simulink model "model"  (R2014a)
(part 3 of 4)

  bus249 : powerlib/Measurements/Load Flow Bus  LConnTagsString=a  ID=bus249  Vbase=150000  Vref=1  Vangle=0  VLF=1  angleLF=0
      settings: AttributesFormatString=|
      | %<ID>
      | %<Vbase>V
      | %<VLF>pu
      | %<angleLF>deg.
      | %<Name>
  bus25 : powerlib/Measurements/Load Flow Bus  LConnTagsString=a  ID=bus25  Vbase=150000  Vref=1  Vangle=0  VLF=1  angleLF=0
      settings: AttributesFormatString=|
      | %<ID>
      | %<Vbase>V
      | %<VLF>pu
      | %<angleLF>deg.
      | %<Name>
  bus250 : powerlib/Measurements/Load Flow Bus  LConnTagsString=a  ID=bus250  Vbase=150000  Vref=1  Vangle=0  VLF=1  angleLF=0
      settings: AttributesFormatString=|
      | %<ID>
      | %<Vbase>V
      | %<VLF>pu
      | %<angleLF>deg.
      | %<Name>
  bus251 : powerlib/Measurements/Load Flow Bus  LConnTagsString=a  ID=bus251  Vbase=150000  Vref=1  Vangle=0  VLF=1  angleLF=0
      settings: AttributesFormatString=|
      | %<ID>
      | %<Vbase>V
      | %<VLF>pu
      | %<angleLF>deg.
      | %<Name>
  bus252 : powerlib/Measurements/Load Flow Bus  LConnTagsString=a  ID=bus252  Vbase=150000  Vref=1  Vangle=0  VLF=1  angleLF=0
      settings: AttributesFormatString=|
      | %<ID>
      | %<Vbase>V
      | %<VLF>pu
      | %<angleLF>deg.
      | %<Name>
  bus253 : powerlib/Measurements/Load Flow Bus  LConnTagsString=a  ID=bus253  Vbase=150000  Vref=1  Vangle=0  VLF=1  angleLF=0
      settings: AttributesFormatString=|
      | %<ID>
      | %<Vbase>V
      | %<VLF>pu
      | %<angleLF>deg.
      | %<Name>
  bus254 : powerlib/Measurements/Load Flow Bus  LConnTagsString=a  ID=bus254  Vbase=150000  Vref=1  Vangle=0  VLF=1  angleLF=0
      settings: AttributesFormatString=|
      | %<ID>
      | %<Vbase>V
      | %<VLF>pu
      | %<angleLF>deg.
      | %<Name>
  bus255 : powerlib/Measurements/Load Flow Bus  LConnTagsString=a  ID=bus255  Vbase=150000  Vref=1  Vangle=0  VLF=1  angleLF=0
      settings: AttributesFormatString=|
      | %<ID>
      | %<Vbase>V
      | %<VLF>pu
      | %<angleLF>deg.
      | %<Name>
  bus256 : powerlib/Measurements/Load Flow Bus  LConnTagsString=a  ID=bus256  Vbase=150000  Vref=1  Vangle=0  VLF=1  angleLF=0
      settings: AttributesFormatString=|
      | %<ID>
      | %<Vbase>V
      | %<VLF>pu
      | %<angleLF>deg.
      | %<Name>
  bus257 : powerlib/Measurements/Load Flow Bus  LConnTagsString=a  ID=bus257  Vbase=150000  Vref=1  Vangle=0  VLF=1  angleLF=0
      settings: AttributesFormatString=|
      | %<ID>
      | %<Vbase>V
      | %<VLF>pu
      | %<angleLF>deg.
      | %<Name>
  bus258 : powerlib/Measurements/Load Flow Bus  LConnTagsString=a  ID=bus258  Vbase=150000  Vref=1  Vangle=0  VLF=1  angleLF=0
      settings: AttributesFormatString=|
      | %<ID>
      | %<Vbase>V
      | %<VLF>pu
      | %<angleLF>deg.
      | %<Name>
  bus259 : powerlib/Measurements/Load Flow Bus  LConnTagsString=a  ID=bus259  Vbase=150000  Vref=1  Vangle=0  VLF=1  angleLF=0
      settings: AttributesFormatString=|
      | %<ID>
      | %<Vbase>V
      | %<VLF>pu
      | %<angleLF>deg.
      | %<Name>
  bus26 : powerlib/Measurements/Load Flow Bus  LConnTagsString=a  ID=bus26  Vbase=150000  Vref=1  Vangle=0  VLF=1  angleLF=0
      settings: AttributesFormatString=|
      | %<ID>
      | %<Vbase>V
      | %<VLF>pu
      | %<angleLF>deg.
      | %<Name>
  bus260 : powerlib/Measurements/Load Flow Bus  LConnTagsString=a  ID=bus260  Vbase=150000  Vref=1  Vangle=0  VLF=1  angleLF=0
      settings: AttributesFormatString=|
      | %<ID>
      | %<Vbase>V
      | %<VLF>pu
      | %<angleLF>deg.
      | %<Name>
  bus261 : powerlib/Measurements/Load Flow Bus  LConnTagsString=a  ID=bus261  Vbase=150000  Vref=1  Vangle=0  VLF=1  angleLF=0
      settings: AttributesFormatString=|
      | %<ID>
      | %<Vbase>V
      | %<VLF>pu
      | %<angleLF>deg.
      | %<Name>
  bus262 : powerlib/Measurements/Load Flow Bus  LConnTagsString=a  ID=bus262  Vbase=150000  Vref=1  Vangle=0  VLF=1  angleLF=0
      settings: AttributesFormatString=|
      | %<ID>
      | %<Vbase>V
      | %<VLF>pu
      | %<angleLF>deg.
      | %<Name>
  bus263 : powerlib/Measurements/Load Flow Bus  LConnTagsString=a  ID=bus263  Vbase=150000  Vref=1  Vangle=0  VLF=1  angleLF=0
      settings: AttributesFormatString=|
      | %<ID>
      | %<Vbase>V
      | %<VLF>pu
      | %<angleLF>deg.
      | %<Name>
  bus264 : powerlib/Measurements/Load Flow Bus  LConnTagsString=a  ID=bus264  Vbase=150000  Vref=1  Vangle=0  VLF=1  angleLF=0
      settings: AttributesFormatString=|
      | %<ID>
      | %<Vbase>V
      | %<VLF>pu
      | %<angleLF>deg.
      | %<Name>
  bus265 : powerlib/Measurements/Load Flow Bus  LConnTagsString=a  ID=bus265  Vbase=150000  Vref=1  Vangle=0  VLF=1  angleLF=0
      settings: AttributesFormatString=|
      | %<ID>
      | %<Vbase>V
      | %<VLF>pu
      | %<angleLF>deg.
      | %<Name>
  bus266 : powerlib/Measurements/Load Flow Bus  LConnTagsString=a  ID=bus266  Vbase=150000  Vref=1  Vangle=0  VLF=1  angleLF=0
      settings: AttributesFormatString=|
      | %<ID>
      | %<Vbase>V
      | %<VLF>pu
      | %<angleLF>deg.
      | %<Name>
  bus267 : powerlib/Measurements/Load Flow Bus  LConnTagsString=a  ID=bus267  Vbase=150000  Vref=1  Vangle=0  VLF=1  angleLF=0
      settings: AttributesFormatString=|
      | %<ID>
      | %<Vbase>V
      | %<VLF>pu
      | %<angleLF>deg.
      | %<Name>
  bus268 : powerlib/Measurements/Load Flow Bus  LConnTagsString=a  ID=bus268  Vbase=150000  Vref=1  Vangle=0  VLF=1  angleLF=0
      settings: AttributesFormatString=|
      | %<ID>
      | %<Vbase>V
      | %<VLF>pu
      | %<angleLF>deg.
      | %<Name>
  bus269 : powerlib/Measurements/Load Flow Bus  LConnTagsString=a  ID=bus269  Vbase=150000  Vref=1  Vangle=0  VLF=1  angleLF=0
      settings: AttributesFormatString=|
      | %<ID>
      | %<Vbase>V
      | %<VLF>pu
      | %<angleLF>deg.
      | %<Name>
  bus27 : powerlib/Measurements/Load Flow Bus  LConnTagsString=a  ID=bus27  Vbase=150000  Vref=1  Vangle=0  VLF=1  angleLF=0
      settings: AttributesFormatString=|
      | %<ID>
      | %<Vbase>V
      | %<VLF>pu
      | %<angleLF>deg.
      | %<Name>
  bus270 : powerlib/Measurements/Load Flow Bus  LConnTagsString=a  ID=bus270  Vbase=150000  Vref=1  Vangle=0  VLF=1  angleLF=0
      settings: AttributesFormatString=|
      | %<ID>
      | %<Vbase>V
      | %<VLF>pu
      | %<angleLF>deg.
      | %<Name>
  bus271 : powerlib/Measurements/Load Flow Bus  LConnTagsString=a  ID=bus271  Vbase=150000  Vref=1  Vangle=0  VLF=1  angleLF=0
      settings: AttributesFormatString=|
      | %<ID>
      | %<Vbase>V
      | %<VLF>pu
      | %<angleLF>deg.
      | %<Name>
  bus272 : powerlib/Measurements/Load Flow Bus  LConnTagsString=a  ID=bus272  Vbase=150000  Vref=1  Vangle=0  VLF=1  angleLF=0
      settings: AttributesFormatString=|
      | %<ID>
      | %<Vbase>V
      | %<VLF>pu
      | %<angleLF>deg.
      | %<Name>
  bus273 : powerlib/Measurements/Load Flow Bus  LConnTagsString=a  ID=bus273  Vbase=150000  Vref=1  Vangle=0  VLF=1  angleLF=0
      settings: AttributesFormatString=|
      | %<ID>
      | %<Vbase>V
      | %<VLF>pu
      | %<angleLF>deg.
      | %<Name>
  bus274 : powerlib/Measurements/Load Flow Bus  LConnTagsString=a  ID=bus274  Vbase=150000  Vref=1  Vangle=0  VLF=1  angleLF=0
      settings: AttributesFormatString=|
      | %<ID>
      | %<Vbase>V
      | %<VLF>pu
      | %<angleLF>deg.
      | %<Name>
  bus275 : powerlib/Measurements/Load Flow Bus  LConnTagsString=a  ID=bus275  Vbase=150000  Vref=1  Vangle=0  VLF=1  angleLF=0
      settings: AttributesFormatString=|
      | %<ID>
      | %<Vbase>V
      | %<VLF>pu
      | %<angleLF>deg.
      | %<Name>
  bus276 : powerlib/Measurements/Load Flow Bus  LConnTagsString=a  ID=bus276  Vbase=150000  Vref=1  Vangle=0  VLF=1  angleLF=0
      settings: AttributesFormatString=|
      | %<ID>
      | %<Vbase>V
      | %<VLF>pu
      | %<angleLF>deg.
      | %<Name>
  bus277 : powerlib/Measurements/Load Flow Bus  LConnTagsString=a  ID=bus277  Vbase=150000  Vref=1  Vangle=0  VLF=1  angleLF=0
      settings: AttributesFormatString=|
      | %<ID>
      | %<Vbase>V
      | %<VLF>pu
      | %<angleLF>deg.
      | %<Name>
  bus278 : powerlib/Measurements/Load Flow Bus  LConnTagsString=a  ID=bus278  Vbase=150000  Vref=1  Vangle=0  VLF=1  angleLF=0
      settings: AttributesFormatString=|
      | %<ID>
      | %<Vbase>V
      | %<VLF>pu
      | %<angleLF>deg.
      | %<Name>
  bus279 : powerlib/Measurements/Load Flow Bus  LConnTagsString=a  ID=bus279  Vbase=150000  Vref=1  Vangle=0  VLF=1  angleLF=0
      settings: AttributesFormatString=|
      | %<ID>
      | %<Vbase>V
      | %<VLF>pu
      | %<angleLF>deg.
      | %<Name>
  bus28 : powerlib/Measurements/Load Flow Bus  LConnTagsString=a  ID=bus28  Vbase=150000  Vref=1  Vangle=0  VLF=1  angleLF=0
      settings: AttributesFormatString=|
      | %<ID>
      | %<Vbase>V
      | %<VLF>pu
      | %<angleLF>deg.
      | %<Name>
  bus280 : powerlib/Measurements/Load Flow Bus  LConnTagsString=a  ID=bus280  Vbase=150000  Vref=1  Vangle=0  VLF=1  angleLF=0
      settings: AttributesFormatString=|
      | %<ID>
      | %<Vbase>V
      | %<VLF>pu
      | %<angleLF>deg.
      | %<Name>
  bus281 : powerlib/Measurements/Load Flow Bus  LConnTagsString=a  ID=bus281  Vbase=150000  Vref=1  Vangle=0  VLF=1  angleLF=0
      settings: AttributesFormatString=|
      | %<ID>
      | %<Vbase>V
      | %<VLF>pu
      | %<angleLF>deg.
      | %<Name>
  bus282 : powerlib/Measurements/Load Flow Bus  LConnTagsString=a  ID=bus282  Vbase=150000  Vref=1  Vangle=0  VLF=1  angleLF=0
      settings: AttributesFormatString=|
      | %<ID>
      | %<Vbase>V
      | %<VLF>pu
      | %<angleLF>deg.
      | %<Name>
  bus283 : powerlib/Measurements/Load Flow Bus  LConnTagsString=a  ID=bus283  Vbase=150000  Vref=1  Vangle=0  VLF=1  angleLF=0
      settings: AttributesFormatString=|
      | %<ID>
      | %<Vbase>V
      | %<VLF>pu
      | %<angleLF>deg.
      | %<Name>
  bus284 : powerlib/Measurements/Load Flow Bus  LConnTagsString=a  ID=bus284  Vbase=150000  Vref=1  Vangle=0  VLF=1  angleLF=0
      settings: AttributesFormatString=|
      | %<ID>
      | %<Vbase>V
      | %<VLF>pu
      | %<angleLF>deg.
      | %<Name>
  bus285 : powerlib/Measurements/Load Flow Bus  LConnTagsString=a  ID=bus285  Vbase=150000  Vref=1  Vangle=0  VLF=1  angleLF=0
      settings: AttributesFormatString=|
      | %<ID>
      | %<Vbase>V
      | %<VLF>pu
      | %<angleLF>deg.
      | %<Name>
  bus286 : powerlib/Measurements/Load Flow Bus  LConnTagsString=a  ID=bus286  Vbase=150000  Vref=1  Vangle=0  VLF=1  angleLF=0
      settings: AttributesFormatString=|
      | %<ID>
      | %<Vbase>V
      | %<VLF>pu
      | %<angleLF>deg.
      | %<Name>
  bus287 : powerlib/Measurements/Load Flow Bus  LConnTagsString=a  ID=bus287  Vbase=150000  Vref=1  Vangle=0  VLF=1  angleLF=0
      settings: AttributesFormatString=|
      | %<ID>
      | %<Vbase>V
      | %<VLF>pu
      | %<angleLF>deg.
      | %<Name>
  bus288 : powerlib/Measurements/Load Flow Bus  LConnTagsString=a  ID=bus288  Vbase=150000  Vref=1  Vangle=0  VLF=1  angleLF=0
      settings: AttributesFormatString=|
      | %<ID>
      | %<Vbase>V
      | %<VLF>pu
      | %<angleLF>deg.
      | %<Name>
  bus289 : powerlib/Measurements/Load Flow Bus  LConnTagsString=a  ID=bus289  Vbase=150000  Vref=1  Vangle=0  VLF=1  angleLF=0
      settings: AttributesFormatString=|
      | %<ID>
      | %<Vbase>V
      | %<VLF>pu
      | %<angleLF>deg.
      | %<Name>
  bus29 : powerlib/Measurements/Load Flow Bus  LConnTagsString=a  ID=bus29  Vbase=150000  Vref=1  Vangle=0  VLF=1  angleLF=0
      settings: AttributesFormatString=|
      | %<ID>
      | %<Vbase>V
      | %<VLF>pu
      | %<angleLF>deg.
      | %<Name>
  bus290 : powerlib/Measurements/Load Flow Bus  LConnTagsString=a  ID=bus290  Vbase=150000  Vref=1  Vangle=0  VLF=1  angleLF=0
      settings: AttributesFormatString=|
      | %<ID>
      | %<Vbase>V
      | %<VLF>pu
      | %<angleLF>deg.
      | %<Name>
  bus291 : powerlib/Measurements/Load Flow Bus  LConnTagsString=a  ID=bus291  Vbase=150000  Vref=1  Vangle=0  VLF=1  angleLF=0
      settings: AttributesFormatString=|
      | %<ID>
      | %<Vbase>V
      | %<VLF>pu
      | %<angleLF>deg.
      | %<Name>
  bus292 : powerlib/Measurements/Load Flow Bus  LConnTagsString=a  ID=bus292  Vbase=150000  Vref=1  Vangle=0  VLF=1  angleLF=0
      settings: AttributesFormatString=|
      | %<ID>
      | %<Vbase>V
      | %<VLF>pu
      | %<angleLF>deg.
      | %<Name>
  bus293 : powerlib/Measurements/Load Flow Bus  LConnTagsString=a  ID=bus293  Vbase=150000  Vref=1  Vangle=0  VLF=1  angleLF=0
      settings: AttributesFormatString=|
      | %<ID>
      | %<Vbase>V
      | %<VLF>pu
      | %<angleLF>deg.
      | %<Name>
  bus294 : powerlib/Measurements/Load Flow Bus  LConnTagsString=a  ID=bus294  Vbase=150000  Vref=1  Vangle=0  VLF=1  angleLF=0
      settings: AttributesFormatString=|
      | %<ID>
      | %<Vbase>V
      | %<VLF>pu
      | %<angleLF>deg.
      | %<Name>
  bus295 : powerlib/Measurements/Load Flow Bus  LConnTagsString=a  ID=bus295  Vbase=150000  Vref=1  Vangle=0  VLF=1  angleLF=0
      settings: AttributesFormatString=|
      | %<ID>
      | %<Vbase>V
      | %<VLF>pu
      | %<angleLF>deg.
      | %<Name>
  bus296 : powerlib/Measurements/Load Flow Bus  LConnTagsString=a  ID=bus296  Vbase=150000  Vref=1  Vangle=0  VLF=1  angleLF=0
      settings: AttributesFormatString=|
      | %<ID>
      | %<Vbase>V
      | %<VLF>pu
      | %<angleLF>deg.
      | %<Name>
  bus297 : powerlib/Measurements/Load Flow Bus  LConnTagsString=a  ID=bus297  Vbase=150000  Vref=1  Vangle=0  VLF=1  angleLF=0
      settings: AttributesFormatString=|
      | %<ID>
      | %<Vbase>V
      | %<VLF>pu
      | %<angleLF>deg.
      | %<Name>
  bus298 : powerlib/Measurements/Load Flow Bus  LConnTagsString=a  ID=bus298  Vbase=150000  Vref=1  Vangle=0  VLF=1  angleLF=0
      settings: AttributesFormatString=|
      | %<ID>
      | %<Vbase>V
      | %<VLF>pu
      | %<angleLF>deg.
      | %<Name>
  bus299 : powerlib/Measurements/Load Flow Bus  LConnTagsString=a  ID=bus299  Vbase=150000  Vref=1  Vangle=0  VLF=1  angleLF=0
      settings: AttributesFormatString=|
      | %<ID>
      | %<Vbase>V
      | %<VLF>pu
      | %<angleLF>deg.
      | %<Name>
  bus3 : powerlib/Measurements/Load Flow Bus  LConnTagsString=a  ID=bus3  Vbase=150000  Vref=1  Vangle=0  VLF=1  angleLF=0
      settings: AttributesFormatString=|
      | %<ID>
      | %<Vbase>V
      | %<VLF>pu
      | %<angleLF>deg.
      | %<Name>
  bus30 : powerlib/Measurements/Load Flow Bus  LConnTagsString=a  ID=bus30  Vbase=150000  Vref=1  Vangle=0  VLF=1  angleLF=0
      settings: AttributesFormatString=|
      | %<ID>
      | %<Vbase>V
      | %<VLF>pu
      | %<angleLF>deg.
      | %<Name>
  bus300 : powerlib/Measurements/Load Flow Bus  LConnTagsString=a  ID=bus300  Vbase=150000  Vref=1  Vangle=0  VLF=1  angleLF=0
      settings: AttributesFormatString=|
      | %<ID>
      | %<Vbase>V
      | %<VLF>pu
      | %<angleLF>deg.
      | %<Name>
  bus301 : powerlib/Measurements/Load Flow Bus  LConnTagsString=a  ID=bus301  Vbase=150000  Vref=1  Vangle=0  VLF=1  angleLF=0
      settings: AttributesFormatString=|
      | %<ID>
      | %<Vbase>V
      | %<VLF>pu
      | %<angleLF>deg.
      | %<Name>
  bus302 : powerlib/Measurements/Load Flow Bus  LConnTagsString=a  ID=bus302  Vbase=150000  Vref=1  Vangle=0  VLF=1  angleLF=0
      settings: AttributesFormatString=|
      | %<ID>
      | %<Vbase>V
      | %<VLF>pu
      | %<angleLF>deg.
      | %<Name>
  bus303 : powerlib/Measurements/Load Flow Bus  LConnTagsString=a  ID=bus303  Vbase=150000  Vref=1  Vangle=0  VLF=1  angleLF=0
      settings: AttributesFormatString=|
      | %<ID>
      | %<Vbase>V
      | %<VLF>pu
      | %<angleLF>deg.
      | %<Name>
  bus304 : powerlib/Measurements/Load Flow Bus  LConnTagsString=a  ID=bus304  Vbase=150000  Vref=1  Vangle=0  VLF=1  angleLF=0
      settings: AttributesFormatString=|
      | %<ID>
      | %<Vbase>V
      | %<VLF>pu
      | %<angleLF>deg.
      | %<Name>
  bus305 : powerlib/Measurements/Load Flow Bus  LConnTagsString=a  ID=bus305  Vbase=150000  Vref=1  Vangle=0  VLF=1  angleLF=0
      settings: AttributesFormatString=|
      | %<ID>
      | %<Vbase>V
      | %<VLF>pu
      | %<angleLF>deg.
      | %<Name>
  bus306 : powerlib/Measurements/Load Flow Bus  LConnTagsString=a  ID=bus306  Vbase=150000  Vref=1  Vangle=0  VLF=1  angleLF=0
      settings: AttributesFormatString=|
      | %<ID>
      | %<Vbase>V
      | %<VLF>pu
      | %<angleLF>deg.
      | %<Name>
  bus307 : powerlib/Measurements/Load Flow Bus  LConnTagsString=a  ID=bus307  Vbase=150000  Vref=1  Vangle=0  VLF=1  angleLF=0
      settings: AttributesFormatString=|
      | %<ID>
      | %<Vbase>V
      | %<VLF>pu
      | %<angleLF>deg.
      | %<Name>
  bus308 : powerlib/Measurements/Load Flow Bus  LConnTagsString=a  ID=bus308  Vbase=150000  Vref=1  Vangle=0  VLF=1  angleLF=0
      settings: AttributesFormatString=|
      | %<ID>
      | %<Vbase>V
      | %<VLF>pu
      | %<angleLF>deg.
      | %<Name>
  bus309 : powerlib/Measurements/Load Flow Bus  LConnTagsString=a  ID=bus309  Vbase=150000  Vref=1  Vangle=0  VLF=1  angleLF=0
      settings: AttributesFormatString=|
      | %<ID>
      | %<Vbase>V
      | %<VLF>pu
      | %<angleLF>deg.
      | %<Name>
  bus31 : powerlib/Measurements/Load Flow Bus  LConnTagsString=a  ID=bus31  Vbase=150000  Vref=1  Vangle=0  VLF=1  angleLF=0
      settings: AttributesFormatString=|
      | %<ID>
      | %<Vbase>V
      | %<VLF>pu
      | %<angleLF>deg.
      | %<Name>
  bus310 : powerlib/Measurements/Load Flow Bus  LConnTagsString=a  ID=bus310  Vbase=150000  Vref=1  Vangle=0  VLF=1  angleLF=0
      settings: AttributesFormatString=|
      | %<ID>
      | %<Vbase>V
      | %<VLF>pu
      | %<angleLF>deg.
      | %<Name>
  bus311 : powerlib/Measurements/Load Flow Bus  LConnTagsString=a  ID=bus311  Vbase=150000  Vref=1  Vangle=0  VLF=1  angleLF=0
      settings: AttributesFormatString=|
      | %<ID>
      | %<Vbase>V
      | %<VLF>pu
      | %<angleLF>deg.
      | %<Name>
  bus312 : powerlib/Measurements/Load Flow Bus  LConnTagsString=a  ID=bus312  Vbase=150000  Vref=1  Vangle=0  VLF=1  angleLF=0
      settings: AttributesFormatString=|
      | %<ID>
      | %<Vbase>V
      | %<VLF>pu
      | %<angleLF>deg.
      | %<Name>
  bus313 : powerlib/Measurements/Load Flow Bus  LConnTagsString=a  ID=bus313  Vbase=150000  Vref=1  Vangle=0  VLF=1  angleLF=0
      settings: AttributesFormatString=|
      | %<ID>
      | %<Vbase>V
      | %<VLF>pu
      | %<angleLF>deg.
      | %<Name>
  bus314 : powerlib/Measurements/Load Flow Bus  LConnTagsString=a  ID=bus314  Vbase=150000  Vref=1  Vangle=0  VLF=1  angleLF=0
      settings: AttributesFormatString=|
      | %<ID>
      | %<Vbase>V
      | %<VLF>pu
      | %<angleLF>deg.
      | %<Name>
  bus315 : powerlib/Measurements/Load Flow Bus  LConnTagsString=a  ID=bus315  Vbase=150000  Vref=1  Vangle=0  VLF=1  angleLF=0
      settings: AttributesFormatString=|
      | %<ID>
      | %<Vbase>V
      | %<VLF>pu
      | %<angleLF>deg.
      | %<Name>
  bus316 : powerlib/Measurements/Load Flow Bus  LConnTagsString=a  ID=bus316  Vbase=150000  Vref=1  Vangle=0  VLF=1  angleLF=0
      settings: AttributesFormatString=|
      | %<ID>
      | %<Vbase>V
      | %<VLF>pu
      | %<angleLF>deg.
      | %<Name>
  bus317 : powerlib/Measurements/Load Flow Bus  LConnTagsString=a  ID=bus317  Vbase=150000  Vref=1  Vangle=0  VLF=1  angleLF=0
      settings: AttributesFormatString=|
      | %<ID>
      | %<Vbase>V
      | %<VLF>pu
      | %<angleLF>deg.
      | %<Name>
  bus318 : powerlib/Measurements/Load Flow Bus  LConnTagsString=a  ID=bus318  Vbase=150000  Vref=1  Vangle=0  VLF=1  angleLF=0
      settings: AttributesFormatString=|
      | %<ID>
      | %<Vbase>V
      | %<VLF>pu
      | %<angleLF>deg.
      | %<Name>
  bus319 : powerlib/Measurements/Load Flow Bus  LConnTagsString=a  ID=bus319  Vbase=150000  Vref=1  Vangle=0  VLF=1  angleLF=0
      settings: AttributesFormatString=|
      | %<ID>
      | %<Vbase>V
      | %<VLF>pu
      | %<angleLF>deg.
      | %<Name>
  bus32 : powerlib/Measurements/Load Flow Bus  LConnTagsString=a  ID=bus32  Vbase=150000  Vref=1  Vangle=0  VLF=1  angleLF=0
      settings: AttributesFormatString=|
      | %<ID>
      | %<Vbase>V
      | %<VLF>pu
      | %<angleLF>deg.
      | %<Name>
  bus320 : powerlib/Measurements/Load Flow Bus  LConnTagsString=a  ID=bus320  Vbase=150000  Vref=1  Vangle=0  VLF=1  angleLF=0
      settings: AttributesFormatString=|
      | %<ID>
      | %<Vbase>V
      | %<VLF>pu
      | %<angleLF>deg.
      | %<Name>
  bus321 : powerlib/Measurements/Load Flow Bus  LConnTagsString=a  ID=bus321  Vbase=150000  Vref=1  Vangle=0  VLF=1  angleLF=0
      settings: AttributesFormatString=|
      | %<ID>
      | %<Vbase>V
      | %<VLF>pu
      | %<angleLF>deg.
      | %<Name>
  bus322 : powerlib/Measurements/Load Flow Bus  LConnTagsString=a  ID=bus322  Vbase=150000  Vref=1  Vangle=0  VLF=1  angleLF=0
      settings: AttributesFormatString=|
      | %<ID>
      | %<Vbase>V
      | %<VLF>pu
      | %<angleLF>deg.
      | %<Name>
  bus323 : powerlib/Measurements/Load Flow Bus  LConnTagsString=a  ID=bus323  Vbase=150000  Vref=1  Vangle=0  VLF=1  angleLF=0
      settings: AttributesFormatString=|
      | %<ID>
      | %<Vbase>V
      | %<VLF>pu
      | %<angleLF>deg.
      | %<Name>
  bus324 : powerlib/Measurements/Load Flow Bus  LConnTagsString=a  ID=bus324  Vbase=150000  Vref=1  Vangle=0  VLF=1  angleLF=0
      settings: AttributesFormatString=|
      | %<ID>
      | %<Vbase>V
      | %<VLF>pu
      | %<angleLF>deg.
      | %<Name>
  bus325 : powerlib/Measurements/Load Flow Bus  LConnTagsString=a  ID=bus325  Vbase=150000  Vref=1  Vangle=0  VLF=1  angleLF=0
      settings: AttributesFormatString=|
      | %<ID>
      | %<Vbase>V
      | %<VLF>pu
      | %<angleLF>deg.
      | %<Name>
  bus326 : powerlib/Measurements/Load Flow Bus  LConnTagsString=a  ID=bus326  Vbase=150000  Vref=1  Vangle=0  VLF=1  angleLF=0
      settings: AttributesFormatString=|
      | %<ID>
      | %<Vbase>V
      | %<VLF>pu
      | %<angleLF>deg.
      | %<Name>
  bus327 : powerlib/Measurements/Load Flow Bus  LConnTagsString=a  ID=bus327  Vbase=150000  Vref=1  Vangle=0  VLF=1  angleLF=0
      settings: AttributesFormatString=|
      | %<ID>
      | %<Vbase>V
      | %<VLF>pu
      | %<angleLF>deg.
      | %<Name>
  bus328 : powerlib/Measurements/Load Flow Bus  LConnTagsString=a  ID=bus328  Vbase=150000  Vref=1  Vangle=0  VLF=1  angleLF=0
      settings: AttributesFormatString=|
      | %<ID>
      | %<Vbase>V
      | %<VLF>pu
      | %<angleLF>deg.
      | %<Name>
  bus329 : powerlib/Measurements/Load Flow Bus  LConnTagsString=a  ID=bus329  Vbase=150000  Vref=1  Vangle=0  VLF=1  angleLF=0
      settings: AttributesFormatString=|
      | %<ID>
      | %<Vbase>V
      | %<VLF>pu
      | %<angleLF>deg.
      | %<Name>
  bus33 : powerlib/Measurements/Load Flow Bus  LConnTagsString=a  ID=bus33  Vbase=150000  Vref=1  Vangle=0  VLF=1  angleLF=0
      settings: AttributesFormatString=|
      | %<ID>
      | %<Vbase>V
      | %<VLF>pu
      | %<angleLF>deg.
      | %<Name>
  bus330 : powerlib/Measurements/Load Flow Bus  LConnTagsString=a  ID=bus330  Vbase=150000  Vref=1  Vangle=0  VLF=1  angleLF=0
      settings: AttributesFormatString=|
      | %<ID>
      | %<Vbase>V
      | %<VLF>pu
      | %<angleLF>deg.
      | %<Name>
  bus331 : powerlib/Measurements/Load Flow Bus  LConnTagsString=a  ID=bus331  Vbase=150000  Vref=1  Vangle=0  VLF=1  angleLF=0
      settings: AttributesFormatString=|
      | %<ID>
      | %<Vbase>V
      | %<VLF>pu
      | %<angleLF>deg.
      | %<Name>
  bus332 : powerlib/Measurements/Load Flow Bus  LConnTagsString=a  ID=bus332  Vbase=150000  Vref=1  Vangle=0  VLF=1  angleLF=0
      settings: AttributesFormatString=|
      | %<ID>
      | %<Vbase>V
      | %<VLF>pu
      | %<angleLF>deg.
      | %<Name>
  bus333 : powerlib/Measurements/Load Flow Bus  LConnTagsString=a  ID=bus333  Vbase=150000  Vref=1  Vangle=0  VLF=1  angleLF=0
      settings: AttributesFormatString=|
      | %<ID>
      | %<Vbase>V
      | %<VLF>pu
      | %<angleLF>deg.
      | %<Name>
  bus334 : powerlib/Measurements/Load Flow Bus  LConnTagsString=a  ID=bus334  Vbase=150000  Vref=1  Vangle=0  VLF=1  angleLF=0
      settings: AttributesFormatString=|
      | %<ID>
      | %<Vbase>V
      | %<VLF>pu
      | %<angleLF>deg.
      | %<Name>
  bus335 : powerlib/Measurements/Load Flow Bus  LConnTagsString=a  ID=bus335  Vbase=150000  Vref=1  Vangle=0  VLF=1  angleLF=0
      settings: AttributesFormatString=|
      | %<ID>
      | %<Vbase>V
      | %<VLF>pu
      | %<angleLF>deg.
      | %<Name>
  bus336 : powerlib/Measurements/Load Flow Bus  LConnTagsString=a  ID=bus336  Vbase=150000  Vref=1  Vangle=0  VLF=1  angleLF=0
      settings: AttributesFormatString=|
      | %<ID>
      | %<Vbase>V
      | %<VLF>pu
      | %<angleLF>deg.
      | %<Name>
  bus337 : powerlib/Measurements/Load Flow Bus  LConnTagsString=a  ID=bus337  Vbase=150000  Vref=1  Vangle=0  VLF=1  angleLF=0
      settings: AttributesFormatString=|
      | %<ID>
      | %<Vbase>V
      | %<VLF>pu
      | %<angleLF>deg.
      | %<Name>
  bus338 : powerlib/Measurements/Load Flow Bus  LConnTagsString=a  ID=bus338  Vbase=150000  Vref=1  Vangle=0  VLF=1  angleLF=0
      settings: AttributesFormatString=|
      | %<ID>
      | %<Vbase>V
      | %<VLF>pu
      | %<angleLF>deg.
      | %<Name>
  bus339 : powerlib/Measurements/Load Flow Bus  LConnTagsString=a  ID=bus339  Vbase=150000  Vref=1  Vangle=0  VLF=1  angleLF=0
      settings: AttributesFormatString=|
      | %<ID>
      | %<Vbase>V
      | %<VLF>pu
      | %<angleLF>deg.
      | %<Name>
  bus34 : powerlib/Measurements/Load Flow Bus  LConnTagsString=a  ID=bus34  Vbase=150000  Vref=1  Vangle=0  VLF=1  angleLF=0
      settings: AttributesFormatString=|
      | %<ID>
      | %<Vbase>V
      | %<VLF>pu
      | %<angleLF>deg.
      | %<Name>
  bus340 : powerlib/Measurements/Load Flow Bus  LConnTagsString=a  ID=bus340  Vbase=150000  Vref=1  Vangle=0  VLF=1  angleLF=0
      settings: AttributesFormatString=|
      | %<ID>
      | %<Vbase>V
      | %<VLF>pu
      | %<angleLF>deg.
      | %<Name>
  bus341 : powerlib/Measurements/Load Flow Bus  LConnTagsString=a  ID=bus341  Vbase=150000  Vref=1  Vangle=0  VLF=1  angleLF=0
      settings: AttributesFormatString=|
      | %<ID>
      | %<Vbase>V
      | %<VLF>pu
      | %<angleLF>deg.
      | %<Name>
  bus342 : powerlib/Measurements/Load Flow Bus  LConnTagsString=a  ID=bus342  Vbase=150000  Vref=1  Vangle=0  VLF=1  angleLF=0
      settings: AttributesFormatString=|
      | %<ID>
      | %<Vbase>V
      | %<VLF>pu
      | %<angleLF>deg.
      | %<Name>
  bus343 : powerlib/Measurements/Load Flow Bus  LConnTagsString=a  ID=bus343  Vbase=150000  Vref=1  Vangle=0  VLF=1  angleLF=0
      settings: AttributesFormatString=|
      | %<ID>
      | %<Vbase>V
      | %<VLF>pu
      | %<angleLF>deg.
      | %<Name>
  bus344 : powerlib/Measurements/Load Flow Bus  LConnTagsString=a  ID=bus344  Vbase=150000  Vref=1  Vangle=0  VLF=1  angleLF=0
      settings: AttributesFormatString=|
      | %<ID>
      | %<Vbase>V
      | %<VLF>pu
      | %<angleLF>deg.
      | %<Name>
  bus345 : powerlib/Measurements/Load Flow Bus  LConnTagsString=a  ID=bus345  Vbase=150000  Vref=1  Vangle=0  VLF=1  angleLF=0
      settings: AttributesFormatString=|
      | %<ID>
      | %<Vbase>V
      | %<VLF>pu
      | %<angleLF>deg.
      | %<Name>
  bus346 : powerlib/Measurements/Load Flow Bus  LConnTagsString=a  ID=bus346  Vbase=150000  Vref=1  Vangle=0  VLF=1  angleLF=0
      settings: AttributesFormatString=|
      | %<ID>
      | %<Vbase>V
      | %<VLF>pu
      | %<angleLF>deg.
      | %<Name>
  bus347 : powerlib/Measurements/Load Flow Bus  LConnTagsString=a  ID=bus347  Vbase=150000  Vref=1  Vangle=0  VLF=1  angleLF=0
      settings: AttributesFormatString=|
      | %<ID>
      | %<Vbase>V
      | %<VLF>pu
      | %<angleLF>deg.
      | %<Name>
  bus348 : powerlib/Measurements/Load Flow Bus  LConnTagsString=a  ID=bus348  Vbase=150000  Vref=1  Vangle=0  VLF=1  angleLF=0
      settings: AttributesFormatString=|
      | %<ID>
      | %<Vbase>V
      | %<VLF>pu
      | %<angleLF>deg.
      | %<Name>
  bus349 : powerlib/Measurements/Load Flow Bus  LConnTagsString=a  ID=bus349  Vbase=150000  Vref=1  Vangle=0  VLF=1  angleLF=0
      settings: AttributesFormatString=|
      | %<ID>
      | %<Vbase>V
      | %<VLF>pu
      | %<angleLF>deg.
      | %<Name>
  bus35 : powerlib/Measurements/Load Flow Bus  LConnTagsString=a  ID=bus35  Vbase=150000  Vref=1  Vangle=0  VLF=1  angleLF=0
      settings: AttributesFormatString=|
      | %<ID>
      | %<Vbase>V
      | %<VLF>pu
      | %<angleLF>deg.
      | %<Name>
  bus350 : powerlib/Measurements/Load Flow Bus  LConnTagsString=a  ID=bus350  Vbase=150000  Vref=1  Vangle=0  VLF=1  angleLF=0
      settings: AttributesFormatString=|
      | %<ID>
      | %<Vbase>V
      | %<VLF>pu
      | %<angleLF>deg.
      | %<Name>
  bus351 : powerlib/Measurements/Load Flow Bus  LConnTagsString=a  ID=bus351  Vbase=150000  Vref=1  Vangle=0  VLF=1  angleLF=0
      settings: AttributesFormatString=|
      | %<ID>
      | %<Vbase>V
      | %<VLF>pu
      | %<angleLF>deg.
      | %<Name>
  bus352 : powerlib/Measurements/Load Flow Bus  LConnTagsString=a  ID=bus352  Vbase=150000  Vref=1  Vangle=0  VLF=1  angleLF=0
      settings: AttributesFormatString=|
      | %<ID>
      | %<Vbase>V
      | %<VLF>pu
      | %<angleLF>deg.
      | %<Name>
  bus353 : powerlib/Measurements/Load Flow Bus  LConnTagsString=a  ID=bus353  Vbase=150000  Vref=1  Vangle=0  VLF=1  angleLF=0
      settings: AttributesFormatString=|
      | %<ID>
      | %<Vbase>V
      | %<VLF>pu
      | %<angleLF>deg.
      | %<Name>
  bus354 : powerlib/Measurements/Load Flow Bus  LConnTagsString=a  ID=bus354  Vbase=150000  Vref=1  Vangle=0  VLF=1  angleLF=0
      settings: AttributesFormatString=|
      | %<ID>
      | %<Vbase>V
      | %<VLF>pu
      | %<angleLF>deg.
      | %<Name>
  bus355 : powerlib/Measurements/Load Flow Bus  LConnTagsString=a  ID=bus355  Vbase=150000  Vref=1  Vangle=0  VLF=1  angleLF=0
      settings: AttributesFormatString=|
      | %<ID>
      | %<Vbase>V
      | %<VLF>pu
      | %<angleLF>deg.
      | %<Name>
  bus356 : powerlib/Measurements/Load Flow Bus  LConnTagsString=a  ID=bus356  Vbase=150000  Vref=1  Vangle=0  VLF=1  angleLF=0
      settings: AttributesFormatString=|
      | %<ID>
      | %<Vbase>V
      | %<VLF>pu
      | %<angleLF>deg.
      | %<Name>
  bus357 : powerlib/Measurements/Load Flow Bus  LConnTagsString=a  ID=bus357  Vbase=150000  Vref=1  Vangle=0  VLF=1  angleLF=0
      settings: AttributesFormatString=|
      | %<ID>
      | %<Vbase>V
      | %<VLF>pu
      | %<angleLF>deg.
      | %<Name>
  bus358 : powerlib/Measurements/Load Flow Bus  LConnTagsString=a  ID=bus358  Vbase=150000  Vref=1  Vangle=0  VLF=1  angleLF=0
      settings: AttributesFormatString=|
      | %<ID>
      | %<Vbase>V
      | %<VLF>pu
      | %<angleLF>deg.
      | %<Name>
  bus359 : powerlib/Measurements/Load Flow Bus  LConnTagsString=a  ID=bus359  Vbase=150000  Vref=1  Vangle=0  VLF=1  angleLF=0
      settings: AttributesFormatString=|
      | %<ID>
      | %<Vbase>V
      | %<VLF>pu
      | %<angleLF>deg.
      | %<Name>
  bus36 : powerlib/Measurements/Load Flow Bus  LConnTagsString=a  ID=bus36  Vbase=150000  Vref=1  Vangle=0  VLF=1  angleLF=0
      settings: AttributesFormatString=|
      | %<ID>
      | %<Vbase>V
      | %<VLF>pu
      | %<angleLF>deg.
      | %<Name>
  bus360 : powerlib/Measurements/Load Flow Bus  LConnTagsString=a  ID=bus360  Vbase=150000  Vref=1  Vangle=0  VLF=1  angleLF=0
      settings: AttributesFormatString=|
      | %<ID>
      | %<Vbase>V
      | %<VLF>pu
      | %<angleLF>deg.
      | %<Name>
  bus361 : powerlib/Measurements/Load Flow Bus  LConnTagsString=a  ID=bus361  Vbase=150000  Vref=1  Vangle=0  VLF=1  angleLF=0
      settings: AttributesFormatString=|
      | %<ID>
      | %<Vbase>V
      | %<VLF>pu
      | %<angleLF>deg.
      | %<Name>
  bus362 : powerlib/Measurements/Load Flow Bus  LConnTagsString=a  ID=bus362  Vbase=150000  Vref=1  Vangle=0  VLF=1  angleLF=0
      settings: AttributesFormatString=|
      | %<ID>
      | %<Vbase>V
      | %<VLF>pu
      | %<angleLF>deg.
      | %<Name>
  bus363 : powerlib/Measurements/Load Flow Bus  LConnTagsString=a  ID=bus363  Vbase=150000  Vref=1  Vangle=0  VLF=1  angleLF=0
      settings: AttributesFormatString=|
      | %<ID>
      | %<Vbase>V
      | %<VLF>pu
      | %<angleLF>deg.
      | %<Name>
  bus364 : powerlib/Measurements/Load Flow Bus  LConnTagsString=a  ID=bus364  Vbase=150000  Vref=1  Vangle=0  VLF=1  angleLF=0
      settings: AttributesFormatString=|
      | %<ID>
      | %<Vbase>V
      | %<VLF>pu
      | %<angleLF>deg.
      | %<Name>
  bus365 : powerlib/Measurements/Load Flow Bus  LConnTagsString=a  ID=bus365  Vbase=150000  Vref=1  Vangle=0  VLF=1  angleLF=0
      settings: AttributesFormatString=|
      | %<ID>
      | %<Vbase>V
      | %<VLF>pu
      | %<angleLF>deg.
      | %<Name>
  bus366 : powerlib/Measurements/Load Flow Bus  LConnTagsString=a  ID=bus366  Vbase=150000  Vref=1  Vangle=0  VLF=1  angleLF=0
      settings: AttributesFormatString=|
      | %<ID>
      | %<Vbase>V
      | %<VLF>pu
      | %<angleLF>deg.
      | %<Name>
  bus367 : powerlib/Measurements/Load Flow Bus  LConnTagsString=a  ID=bus367  Vbase=150000  Vref=1  Vangle=0  VLF=1  angleLF=0
      settings: AttributesFormatString=|
      | %<ID>
      | %<Vbase>V
      | %<VLF>pu
      | %<angleLF>deg.
      | %<Name>
  bus368 : powerlib/Measurements/Load Flow Bus  LConnTagsString=a  ID=bus368  Vbase=150000  Vref=1  Vangle=0  VLF=1  angleLF=0
      settings: AttributesFormatString=|
      | %<ID>
      | %<Vbase>V
      | %<VLF>pu
      | %<angleLF>deg.
      | %<Name>
  bus369 : powerlib/Measurements/Load Flow Bus  LConnTagsString=a  ID=bus369  Vbase=150000  Vref=1  Vangle=0  VLF=1  angleLF=0
      settings: AttributesFormatString=|
      | %<ID>
      | %<Vbase>V
      | %<VLF>pu
      | %<angleLF>deg.
      | %<Name>
  bus37 : powerlib/Measurements/Load Flow Bus  LConnTagsString=a  ID=bus37  Vbase=150000  Vref=1  Vangle=0  VLF=1  angleLF=0
      settings: AttributesFormatString=|
      | %<ID>
      | %<Vbase>V
      | %<VLF>pu
      | %<angleLF>deg.
      | %<Name>
  bus370 : powerlib/Measurements/Load Flow Bus  LConnTagsString=a  ID=bus370  Vbase=150000  Vref=1  Vangle=0  VLF=1  angleLF=0
      settings: AttributesFormatString=|
      | %<ID>
      | %<Vbase>V
      | %<VLF>pu
      | %<angleLF>deg.
      | %<Name>
  bus371 : powerlib/Measurements/Load Flow Bus  LConnTagsString=a  ID=bus371  Vbase=150000  Vref=1  Vangle=0  VLF=1  angleLF=0
      settings: AttributesFormatString=|
      | %<ID>
      | %<Vbase>V
      | %<VLF>pu
      | %<angleLF>deg.
      | %<Name>
  bus372 : powerlib/Measurements/Load Flow Bus  LConnTagsString=a  ID=bus372  Vbase=150000  Vref=1  Vangle=0  VLF=1  angleLF=0
      settings: AttributesFormatString=|
      | %<ID>
      | %<Vbase>V
      | %<VLF>pu
      | %<angleLF>deg.
      | %<Name>
  bus373 : powerlib/Measurements/Load Flow Bus  LConnTagsString=a  ID=bus373  Vbase=150000  Vref=1  Vangle=0  VLF=1  angleLF=0
      settings: AttributesFormatString=|
      | %<ID>
      | %<Vbase>V
      | %<VLF>pu
      | %<angleLF>deg.
      | %<Name>
  bus374 : powerlib/Measurements/Load Flow Bus  LConnTagsString=a  ID=bus374  Vbase=150000  Vref=1  Vangle=0  VLF=1  angleLF=0
      settings: AttributesFormatString=|
      | %<ID>
      | %<Vbase>V
      | %<VLF>pu
      | %<angleLF>deg.
      | %<Name>
  bus375 : powerlib/Measurements/Load Flow Bus  LConnTagsString=a  ID=bus375  Vbase=150000  Vref=1  Vangle=0  VLF=1  angleLF=0
      settings: AttributesFormatString=|
      | %<ID>
      | %<Vbase>V
      | %<VLF>pu
      | %<angleLF>deg.
      | %<Name>
  bus376 : powerlib/Measurements/Load Flow Bus  LConnTagsString=a  ID=bus376  Vbase=150000  Vref=1  Vangle=0  VLF=1  angleLF=0
      settings: AttributesFormatString=|
      | %<ID>
      | %<Vbase>V
      | %<VLF>pu
      | %<angleLF>deg.
      | %<Name>
  bus377 : powerlib/Measurements/Load Flow Bus  LConnTagsString=a  ID=bus377  Vbase=150000  Vref=1  Vangle=0  VLF=1  angleLF=0
      settings: AttributesFormatString=|
      | %<ID>
      | %<Vbase>V
      | %<VLF>pu
      | %<angleLF>deg.
      | %<Name>
  bus378 : powerlib/Measurements/Load Flow Bus  LConnTagsString=a  ID=bus378  Vbase=150000  Vref=1  Vangle=0  VLF=1  angleLF=0
      settings: AttributesFormatString=|
      | %<ID>
      | %<Vbase>V
      | %<VLF>pu
      | %<angleLF>deg.
      | %<Name>
  bus379 : powerlib/Measurements/Load Flow Bus  LConnTagsString=a  ID=bus379  Vbase=150000  Vref=1  Vangle=0  VLF=1  angleLF=0
      settings: AttributesFormatString=|
      | %<ID>
      | %<Vbase>V
      | %<VLF>pu
      | %<angleLF>deg.
      | %<Name>
  bus38 : powerlib/Measurements/Load Flow Bus  LConnTagsString=a  ID=bus38  Vbase=150000  Vref=1  Vangle=0  VLF=1  angleLF=0
      settings: AttributesFormatString=|
      | %<ID>
      | %<Vbase>V
      | %<VLF>pu
      | %<angleLF>deg.
      | %<Name>
  bus380 : powerlib/Measurements/Load Flow Bus  LConnTagsString=a  ID=bus380  Vbase=150000  Vref=1  Vangle=0  VLF=1  angleLF=0
      settings: AttributesFormatString=|
      | %<ID>
      | %<Vbase>V
      | %<VLF>pu
      | %<angleLF>deg.
      | %<Name>
  bus381 : powerlib/Measurements/Load Flow Bus  LConnTagsString=a  ID=bus381  Vbase=150000  Vref=1  Vangle=0  VLF=1  angleLF=0
      settings: AttributesFormatString=|
      | %<ID>
      | %<Vbase>V
      | %<VLF>pu
      | %<angleLF>deg.
      | %<Name>
  bus382 : powerlib/Measurements/Load Flow Bus  LConnTagsString=a  ID=bus382  Vbase=150000  Vref=1  Vangle=0  VLF=1  angleLF=0
      settings: AttributesFormatString=|
      | %<ID>
      | %<Vbase>V
      | %<VLF>pu
      | %<angleLF>deg.
      | %<Name>
  bus383 : powerlib/Measurements/Load Flow Bus  LConnTagsString=a  ID=bus383  Vbase=500000  Vref=1  Vangle=0  VLF=1  angleLF=0
      settings: AttributesFormatString=|
      | %<ID>
      | %<Vbase>V
      | %<VLF>pu
      | %<angleLF>deg.
      | %<Name>
  bus384 : powerlib/Measurements/Load Flow Bus  LConnTagsString=a  ID=bus384  Vbase=500000  Vref=1  Vangle=0  VLF=1  angleLF=0
      settings: AttributesFormatString=|
      | %<ID>
      | %<Vbase>V
      | %<VLF>pu
      | %<angleLF>deg.
      | %<Name>
  bus385 : powerlib/Measurements/Load Flow Bus  LConnTagsString=a  ID=bus385  Vbase=500000  Vref=1  Vangle=0  VLF=1  angleLF=0
      settings: AttributesFormatString=|
      | %<ID>
      | %<Vbase>V
      | %<VLF>pu
      | %<angleLF>deg.
      | %<Name>
  bus386 : powerlib/Measurements/Load Flow Bus  LConnTagsString=a  ID=bus386  Vbase=500000  Vref=1  Vangle=0  VLF=1  angleLF=0
      settings: AttributesFormatString=|
      | %<ID>
      | %<Vbase>V
      | %<VLF>pu
      | %<angleLF>deg.
      | %<Name>
  bus387 : powerlib/Measurements/Load Flow Bus  LConnTagsString=a  ID=bus387  Vbase=500000  Vref=1  Vangle=0  VLF=1  angleLF=0
      settings: AttributesFormatString=|
      | %<ID>
      | %<Vbase>V
      | %<VLF>pu
      | %<angleLF>deg.
      | %<Name>
  bus388 : powerlib/Measurements/Load Flow Bus  LConnTagsString=a  ID=bus388  Vbase=500000  Vref=1  Vangle=0  VLF=1  angleLF=0
      settings: AttributesFormatString=|
      | %<ID>
      | %<Vbase>V
      | %<VLF>pu
      | %<angleLF>deg.
      | %<Name>
  bus389 : powerlib/Measurements/Load Flow Bus  LConnTagsString=a  ID=bus389  Vbase=500000  Vref=1  Vangle=0  VLF=1  angleLF=0
      settings: AttributesFormatString=|
      | %<ID>
      | %<Vbase>V
      | %<VLF>pu
      | %<angleLF>deg.
      | %<Name>
  bus39 : powerlib/Measurements/Load Flow Bus  LConnTagsString=a  ID=bus39  Vbase=150000  Vref=1  Vangle=0  VLF=1  angleLF=0
      settings: AttributesFormatString=|
      | %<ID>
      | %<Vbase>V
      | %<VLF>pu
      | %<angleLF>deg.
      | %<Name>
  bus390 : powerlib/Measurements/Load Flow Bus  LConnTagsString=a  ID=bus390  Vbase=500000  Vref=1  Vangle=0  VLF=1  angleLF=0
      settings: AttributesFormatString=|
      | %<ID>
      | %<Vbase>V
      | %<VLF>pu
      | %<angleLF>deg.
      | %<Name>
  bus391 : powerlib/Measurements/Load Flow Bus  LConnTagsString=a  ID=bus391  Vbase=500000  Vref=1  Vangle=0  VLF=1  angleLF=0
      settings: AttributesFormatString=|
      | %<ID>
      | %<Vbase>V
      | %<VLF>pu
      | %<angleLF>deg.
      | %<Name>
  bus392 : powerlib/Measurements/Load Flow Bus  LConnTagsString=a  ID=bus392  Vbase=500000  Vref=1  Vangle=0  VLF=1  angleLF=0
      settings: AttributesFormatString=|
      | %<ID>
      | %<Vbase>V
      | %<VLF>pu
      | %<angleLF>deg.
      | %<Name>
  bus393 : powerlib/Measurements/Load Flow Bus  LConnTagsString=a  ID=bus393  Vbase=500000  Vref=1  Vangle=0  VLF=1  angleLF=0
      settings: AttributesFormatString=|
      | %<ID>
      | %<Vbase>V
      | %<VLF>pu
      | %<angleLF>deg.
      | %<Name>
  bus394 : powerlib/Measurements/Load Flow Bus  LConnTagsString=a  ID=bus394  Vbase=500000  Vref=1  Vangle=0  VLF=1  angleLF=0
      settings: AttributesFormatString=|
      | %<ID>
      | %<Vbase>V
      | %<VLF>pu
      | %<angleLF>deg.
      | %<Name>
  bus4 : powerlib/Measurements/Load Flow Bus  LConnTagsString=a  ID=bus4  Vbase=150000  Vref=1  Vangle=0  VLF=1  angleLF=0
      settings: AttributesFormatString=|
      | %<ID>
      | %<Vbase>V
      | %<VLF>pu
      | %<angleLF>deg.
      | %<Name>
  bus40 : powerlib/Measurements/Load Flow Bus  LConnTagsString=a  ID=bus40  Vbase=150000  Vref=1  Vangle=0  VLF=1  angleLF=0
      settings: AttributesFormatString=|
      | %<ID>
      | %<Vbase>V
      | %<VLF>pu
      | %<angleLF>deg.
      | %<Name>
  bus41 : powerlib/Measurements/Load Flow Bus  LConnTagsString=a  ID=bus41  Vbase=150000  Vref=1  Vangle=0  VLF=1  angleLF=0
      settings: AttributesFormatString=|
      | %<ID>
      | %<Vbase>V
      | %<VLF>pu
      | %<angleLF>deg.
      | %<Name>
  bus42 : powerlib/Measurements/Load Flow Bus  LConnTagsString=a  ID=bus42  Vbase=150000  Vref=1  Vangle=0  VLF=1  angleLF=0
      settings: AttributesFormatString=|
      | %<ID>
      | %<Vbase>V
      | %<VLF>pu
      | %<angleLF>deg.
      | %<Name>
  bus43 : powerlib/Measurements/Load Flow Bus  LConnTagsString=a  ID=bus43  Vbase=150000  Vref=1  Vangle=0  VLF=1  angleLF=0
      settings: AttributesFormatString=|
      | %<ID>
      | %<Vbase>V
      | %<VLF>pu
      | %<angleLF>deg.
      | %<Name>
  bus44 : powerlib/Measurements/Load Flow Bus  LConnTagsString=a  ID=bus44  Vbase=150000  Vref=1  Vangle=0  VLF=1  angleLF=0
      settings: AttributesFormatString=|
      | %<ID>
      | %<Vbase>V
      | %<VLF>pu
      | %<angleLF>deg.
      | %<Name>
  bus45 : powerlib/Measurements/Load Flow Bus  LConnTagsString=a  ID=bus45  Vbase=150000  Vref=1  Vangle=0  VLF=1  angleLF=0
      settings: AttributesFormatString=|
      | %<ID>
      | %<Vbase>V
      | %<VLF>pu
      | %<angleLF>deg.
      | %<Name>
  bus46 : powerlib/Measurements/Load Flow Bus  LConnTagsString=a  ID=bus46  Vbase=150000  Vref=1  Vangle=0  VLF=1  angleLF=0
      settings: AttributesFormatString=|
      | %<ID>
      | %<Vbase>V
      | %<VLF>pu
      | %<angleLF>deg.
      | %<Name>
  bus47 : powerlib/Measurements/Load Flow Bus  LConnTagsString=a  ID=bus47  Vbase=150000  Vref=1  Vangle=0  VLF=1  angleLF=0
      settings: AttributesFormatString=|
      | %<ID>
      | %<Vbase>V
      | %<VLF>pu
      | %<angleLF>deg.
      | %<Name>
  bus48 : powerlib/Measurements/Load Flow Bus  LConnTagsString=a  ID=bus48  Vbase=150000  Vref=1  Vangle=0  VLF=1  angleLF=0
      settings: AttributesFormatString=|
      | %<ID>
      | %<Vbase>V
      | %<VLF>pu
      | %<angleLF>deg.
      | %<Name>
  bus49 : powerlib/Measurements/Load Flow Bus  LConnTagsString=a  ID=bus49  Vbase=150000  Vref=1  Vangle=0  VLF=1  angleLF=0
      settings: AttributesFormatString=|
      | %<ID>
      | %<Vbase>V
      | %<VLF>pu
      | %<angleLF>deg.
      | %<Name>
  bus5 : powerlib/Measurements/Load Flow Bus  LConnTagsString=a  ID=bus5  Vbase=150000  Vref=1  Vangle=0  VLF=1  angleLF=0
      settings: AttributesFormatString=|
      | %<ID>
      | %<Vbase>V
      | %<VLF>pu
      | %<angleLF>deg.
      | %<Name>
  bus50 : powerlib/Measurements/Load Flow Bus  LConnTagsString=a  ID=bus50  Vbase=150000  Vref=1  Vangle=0  VLF=1  angleLF=0
      settings: AttributesFormatString=|
      | %<ID>
      | %<Vbase>V
      | %<VLF>pu
      | %<angleLF>deg.
      | %<Name>
  bus51 : powerlib/Measurements/Load Flow Bus  LConnTagsString=a  ID=bus51  Vbase=150000  Vref=1  Vangle=0  VLF=1  angleLF=0
      settings: AttributesFormatString=|
      | %<ID>
      | %<Vbase>V
      | %<VLF>pu
      | %<angleLF>deg.
      | %<Name>
  bus52 : powerlib/Measurements/Load Flow Bus  LConnTagsString=a  ID=bus52  Vbase=150000  Vref=1  Vangle=0  VLF=1  angleLF=0
      settings: AttributesFormatString=|
      | %<ID>
      | %<Vbase>V
      | %<VLF>pu
      | %<angleLF>deg.
      | %<Name>
  bus53 : powerlib/Measurements/Load Flow Bus  LConnTagsString=a  ID=bus53  Vbase=150000  Vref=1  Vangle=0  VLF=1  angleLF=0
      settings: AttributesFormatString=|
      | %<ID>
      | %<Vbase>V
      | %<VLF>pu
      | %<angleLF>deg.
      | %<Name>
  bus54 : powerlib/Measurements/Load Flow Bus  LConnTagsString=a  ID=bus54  Vbase=150000  Vref=1  Vangle=0  VLF=1  angleLF=0
      settings: AttributesFormatString=|
      | %<ID>
      | %<Vbase>V
      | %<VLF>pu
      | %<angleLF>deg.
      | %<Name>
  bus55 : powerlib/Measurements/Load Flow Bus  LConnTagsString=a  ID=bus55  Vbase=150000  Vref=1  Vangle=0  VLF=1  angleLF=0
      settings: AttributesFormatString=|
      | %<ID>
      | %<Vbase>V
      | %<VLF>pu
      | %<angleLF>deg.
      | %<Name>
  bus56 : powerlib/Measurements/Load Flow Bus  LConnTagsString=a  ID=bus56  Vbase=150000  Vref=1  Vangle=0  VLF=1  angleLF=0
      settings: AttributesFormatString=|
      | %<ID>
      | %<Vbase>V
      | %<VLF>pu
      | %<angleLF>deg.
      | %<Name>
  bus57 : powerlib/Measurements/Load Flow Bus  LConnTagsString=a  ID=bus57  Vbase=150000  Vref=1  Vangle=0  VLF=1  angleLF=0
      settings: AttributesFormatString=|
      | %<ID>
      | %<Vbase>V
      | %<VLF>pu
      | %<angleLF>deg.
      | %<Name>
  bus58 : powerlib/Measurements/Load Flow Bus  LConnTagsString=a  ID=bus58  Vbase=150000  Vref=1  Vangle=0  VLF=1  angleLF=0
      settings: AttributesFormatString=|
      | %<ID>
      | %<Vbase>V
      | %<VLF>pu
      | %<angleLF>deg.
      | %<Name>
  bus59 : powerlib/Measurements/Load Flow Bus  LConnTagsString=a  ID=bus59  Vbase=150000  Vref=1  Vangle=0  VLF=1  angleLF=0
      settings: AttributesFormatString=|
      | %<ID>
      | %<Vbase>V
      | %<VLF>pu
      | %<angleLF>deg.
      | %<Name>
  bus6 : powerlib/Measurements/Load Flow Bus  LConnTagsString=a  ID=bus6  Vbase=150000  Vref=1  Vangle=0  VLF=1  angleLF=0
      settings: AttributesFormatString=|
      | %<ID>
      | %<Vbase>V
      | %<VLF>pu
      | %<angleLF>deg.
      | %<Name>
  bus60 : powerlib/Measurements/Load Flow Bus  LConnTagsString=a  ID=bus60  Vbase=150000  Vref=1  Vangle=0  VLF=1  angleLF=0
      settings: AttributesFormatString=|
      | %<ID>
      | %<Vbase>V
      | %<VLF>pu
      | %<angleLF>deg.
      | %<Name>
  bus61 : powerlib/Measurements/Load Flow Bus  LConnTagsString=a  ID=bus61  Vbase=150000  Vref=1  Vangle=0  VLF=1  angleLF=0
      settings: AttributesFormatString=|
      | %<ID>
      | %<Vbase>V
      | %<VLF>pu
      | %<angleLF>deg.
      | %<Name>
  bus62 : powerlib/Measurements/Load Flow Bus  LConnTagsString=a  ID=bus62  Vbase=150000  Vref=1  Vangle=0  VLF=1  angleLF=0
      settings: AttributesFormatString=|
      | %<ID>
      | %<Vbase>V
      | %<VLF>pu
      | %<angleLF>deg.
      | %<Name>
  bus63 : powerlib/Measurements/Load Flow Bus  LConnTagsString=a  ID=bus63  Vbase=150000  Vref=1  Vangle=0  VLF=1  angleLF=0
      settings: AttributesFormatString=|
      | %<ID>
      | %<Vbase>V
      | %<VLF>pu
      | %<angleLF>deg.
      | %<Name>
  bus64 : powerlib/Measurements/Load Flow Bus  LConnTagsString=a  ID=bus64  Vbase=150000  Vref=1  Vangle=0  VLF=1  angleLF=0
      settings: AttributesFormatString=|
      | %<ID>
      | %<Vbase>V
      | %<VLF>pu
      | %<angleLF>deg.
      | %<Name>
  bus65 : powerlib/Measurements/Load Flow Bus  LConnTagsString=a  ID=bus65  Vbase=150000  Vref=1  Vangle=0  VLF=1  angleLF=0
      settings: AttributesFormatString=|
      | %<ID>
      | %<Vbase>V
      | %<VLF>pu
      | %<angleLF>deg.
      | %<Name>
  bus66 : powerlib/Measurements/Load Flow Bus  LConnTagsString=a  ID=bus66  Vbase=150000  Vref=1  Vangle=0  VLF=1  angleLF=0
      settings: AttributesFormatString=|
      | %<ID>
      | %<Vbase>V
      | %<VLF>pu
      | %<angleLF>deg.
      | %<Name>
  bus67 : powerlib/Measurements/Load Flow Bus  LConnTagsString=a  ID=bus67  Vbase=150000  Vref=1  Vangle=0  VLF=1  angleLF=0
      settings: AttributesFormatString=|
      | %<ID>
      | %<Vbase>V
      | %<VLF>pu
      | %<angleLF>deg.
      | %<Name>
  bus68 : powerlib/Measurements/Load Flow Bus  LConnTagsString=a  ID=bus68  Vbase=150000  Vref=1  Vangle=0  VLF=1  angleLF=0
      settings: AttributesFormatString=|
      | %<ID>
      | %<Vbase>V
      | %<VLF>pu
      | %<angleLF>deg.
      | %<Name>
  bus69 : powerlib/Measurements/Load Flow Bus  LConnTagsString=a  ID=bus69  Vbase=150000  Vref=1  Vangle=0  VLF=1  angleLF=0
      settings: AttributesFormatString=|
      | %<ID>
      | %<Vbase>V
      | %<VLF>pu
      | %<angleLF>deg.
      | %<Name>
  bus7 : powerlib/Measurements/Load Flow Bus  LConnTagsString=a  ID=bus7  Vbase=150000  Vref=1  Vangle=0  VLF=1  angleLF=0
      settings: AttributesFormatString=|
      | %<ID>
      | %<Vbase>V
      | %<VLF>pu
      | %<angleLF>deg.
      | %<Name>
  bus70 : powerlib/Measurements/Load Flow Bus  LConnTagsString=a  ID=bus70  Vbase=150000  Vref=1  Vangle=0  VLF=1  angleLF=0
      settings: AttributesFormatString=|
      | %<ID>
      | %<Vbase>V
      | %<VLF>pu
      | %<angleLF>deg.
      | %<Name>
  bus71 : powerlib/Measurements/Load Flow Bus  LConnTagsString=a  ID=bus71  Vbase=150000  Vref=1  Vangle=0  VLF=1  angleLF=0
      settings: AttributesFormatString=|
      | %<ID>
      | %<Vbase>V
      | %<VLF>pu
      | %<angleLF>deg.
      | %<Name>
  bus72 : powerlib/Measurements/Load Flow Bus  LConnTagsString=a  ID=bus72  Vbase=150000  Vref=1  Vangle=0  VLF=1  angleLF=0
      settings: AttributesFormatString=|
      | %<ID>
      | %<Vbase>V
      | %<VLF>pu
      | %<angleLF>deg.
      | %<Name>
  bus73 : powerlib/Measurements/Load Flow Bus  LConnTagsString=a  ID=bus73  Vbase=150000  Vref=1  Vangle=0  VLF=1  angleLF=0
      settings: AttributesFormatString=|
      | %<ID>
      | %<Vbase>V
      | %<VLF>pu
      | %<angleLF>deg.
      | %<Name>
  bus74 : powerlib/Measurements/Load Flow Bus  LConnTagsString=a  ID=bus74  Vbase=150000  Vref=1  Vangle=0  VLF=1  angleLF=0
      settings: AttributesFormatString=|
      | %<ID>
      | %<Vbase>V
      | %<VLF>pu
      | %<angleLF>deg.
      | %<Name>
  bus75 : powerlib/Measurements/Load Flow Bus  LConnTagsString=a  ID=bus75  Vbase=150000  Vref=1  Vangle=0  VLF=1  angleLF=0
      settings: AttributesFormatString=|
      | %<ID>
      | %<Vbase>V
      | %<VLF>pu
      | %<angleLF>deg.
      | %<Name>
  bus76 : powerlib/Measurements/Load Flow Bus  LConnTagsString=a  ID=bus76  Vbase=150000  Vref=1  Vangle=0  VLF=1  angleLF=0
      settings: AttributesFormatString=|
      | %<ID>
      | %<Vbase>V
      | %<VLF>pu
      | %<angleLF>deg.
      | %<Name>
  bus77 : powerlib/Measurements/Load Flow Bus  LConnTagsString=a  ID=bus77  Vbase=150000  Vref=1  Vangle=0  VLF=1  angleLF=0
      settings: AttributesFormatString=|
      | %<ID>
      | %<Vbase>V
      | %<VLF>pu
      | %<angleLF>deg.
      | %<Name>
  bus78 : powerlib/Measurements/Load Flow Bus  LConnTagsString=a  ID=bus78  Vbase=150000  Vref=1  Vangle=0  VLF=1  angleLF=0
      settings: AttributesFormatString=|
      | %<ID>
      | %<Vbase>V
      | %<VLF>pu
      | %<angleLF>deg.
      | %<Name>
  bus79 : powerlib/Measurements/Load Flow Bus  LConnTagsString=a  ID=bus79  Vbase=150000  Vref=1  Vangle=0  VLF=1  angleLF=0
      settings: AttributesFormatString=|
      | %<ID>
      | %<Vbase>V
      | %<VLF>pu
      | %<angleLF>deg.
      | %<Name>
  bus8 : powerlib/Measurements/Load Flow Bus  LConnTagsString=a  ID=bus8  Vbase=150000  Vref=1  Vangle=0  VLF=1  angleLF=0
      settings: AttributesFormatString=|
      | %<ID>
      | %<Vbase>V
      | %<VLF>pu
      | %<angleLF>deg.
      | %<Name>
  bus80 : powerlib/Measurements/Load Flow Bus  LConnTagsString=a  ID=bus80  Vbase=150000  Vref=1  Vangle=0  VLF=1  angleLF=0
      settings: AttributesFormatString=|
      | %<ID>
      | %<Vbase>V
      | %<VLF>pu
      | %<angleLF>deg.
      | %<Name>
  bus81 : powerlib/Measurements/Load Flow Bus  LConnTagsString=a  ID=bus81  Vbase=150000  Vref=1  Vangle=0  VLF=1  angleLF=0
      settings: AttributesFormatString=|
      | %<ID>
      | %<Vbase>V
      | %<VLF>pu
      | %<angleLF>deg.
      | %<Name>
  bus82 : powerlib/Measurements/Load Flow Bus  LConnTagsString=a  ID=bus82  Vbase=150000  Vref=1  Vangle=0  VLF=1  angleLF=0
      settings: AttributesFormatString=|
      | %<ID>
      | %<Vbase>V
      | %<VLF>pu
      | %<angleLF>deg.
      | %<Name>
  bus83 : powerlib/Measurements/Load Flow Bus  LConnTagsString=a  ID=bus83  Vbase=150000  Vref=1  Vangle=0  VLF=1  angleLF=0
      settings: AttributesFormatString=|
      | %<ID>
      | %<Vbase>V
      | %<VLF>pu
      | %<angleLF>deg.
      | %<Name>
  bus84 : powerlib/Measurements/Load Flow Bus  LConnTagsString=a  ID=bus84  Vbase=150000  Vref=1  Vangle=0  VLF=1  angleLF=0
      settings: AttributesFormatString=|
      | %<ID>
      | %<Vbase>V
      | %<VLF>pu
      | %<angleLF>deg.
      | %<Name>
  bus85 : powerlib/Measurements/Load Flow Bus  LConnTagsString=a  ID=bus85  Vbase=150000  Vref=1  Vangle=0  VLF=1  angleLF=0
      settings: AttributesFormatString=|
      | %<ID>
      | %<Vbase>V
      | %<VLF>pu
      | %<angleLF>deg.
      | %<Name>
  bus86 : powerlib/Measurements/Load Flow Bus  LConnTagsString=a  ID=bus86  Vbase=150000  Vref=1  Vangle=0  VLF=1  angleLF=0
      settings: AttributesFormatString=|
      | %<ID>
      | %<Vbase>V
      | %<VLF>pu
      | %<angleLF>deg.
      | %<Name>
  bus87 : powerlib/Measurements/Load Flow Bus  LConnTagsString=a  ID=bus87  Vbase=150000  Vref=1  Vangle=0  VLF=1  angleLF=0
      settings: AttributesFormatString=|
      | %<ID>
      | %<Vbase>V
      | %<VLF>pu
      | %<angleLF>deg.
      | %<Name>
  bus88 : powerlib/Measurements/Load Flow Bus  LConnTagsString=a  ID=bus88  Vbase=150000  Vref=1  Vangle=0  VLF=1  angleLF=0
      settings: AttributesFormatString=|
      | %<ID>
      | %<Vbase>V
      | %<VLF>pu
      | %<angleLF>deg.
      | %<Name>
  bus89 : powerlib/Measurements/Load Flow Bus  LConnTagsString=a  ID=bus89  Vbase=150000  Vref=1  Vangle=0  VLF=1  angleLF=0
      settings: AttributesFormatString=|
      | %<ID>
      | %<Vbase>V
      | %<VLF>pu
      | %<angleLF>deg.
      | %<Name>
  bus9 : powerlib/Measurements/Load Flow Bus  LConnTagsString=a  ID=bus9  Vbase=150000  Vref=1  Vangle=0  VLF=1  angleLF=0
      settings: AttributesFormatString=|
      | %<ID>
      | %<Vbase>V
      | %<VLF>pu
      | %<angleLF>deg.
      | %<Name>
  bus90 : powerlib/Measurements/Load Flow Bus  LConnTagsString=a  ID=bus90  Vbase=150000  Vref=1  Vangle=0  VLF=1  angleLF=0
      settings: AttributesFormatString=|
      | %<ID>
      | %<Vbase>V
      | %<VLF>pu
      | %<angleLF>deg.
      | %<Name>
  bus91 : powerlib/Measurements/Load Flow Bus  LConnTagsString=a  ID=bus91  Vbase=150000  Vref=1  Vangle=0  VLF=1  angleLF=0
      settings: AttributesFormatString=|
      | %<ID>
      | %<Vbase>V
      | %<VLF>pu
      | %<angleLF>deg.
      | %<Name>
  bus92 : powerlib/Measurements/Load Flow Bus  LConnTagsString=a  ID=bus92  Vbase=150000  Vref=1  Vangle=0  VLF=1  angleLF=0
      settings: AttributesFormatString=|
      | %<ID>
      | %<Vbase>V
      | %<VLF>pu
      | %<angleLF>deg.
      | %<Name>
  bus93 : powerlib/Measurements/Load Flow Bus  LConnTagsString=a  ID=bus93  Vbase=150000  Vref=1  Vangle=0  VLF=1  angleLF=0
      settings: AttributesFormatString=|
      | %<ID>
      | %<Vbase>V
      | %<VLF>pu
      | %<angleLF>deg.
      | %<Name>
  bus94 : powerlib/Measurements/Load Flow Bus  LConnTagsString=a  ID=bus94  Vbase=150000  Vref=1  Vangle=0  VLF=1  angleLF=0
      settings: AttributesFormatString=|
      | %<ID>
      | %<Vbase>V
      | %<VLF>pu
      | %<angleLF>deg.
      | %<Name>
  bus95 : powerlib/Measurements/Load Flow Bus  LConnTagsString=a  ID=bus95  Vbase=150000  Vref=1  Vangle=0  VLF=1  angleLF=0
      settings: AttributesFormatString=|
      | %<ID>
      | %<Vbase>V
      | %<VLF>pu
      | %<angleLF>deg.
      | %<Name>
  bus96 : powerlib/Measurements/Load Flow Bus  LConnTagsString=a  ID=bus96  Vbase=150000  Vref=1  Vangle=0  VLF=1  angleLF=0
      settings: AttributesFormatString=|
      | %<ID>
      | %<Vbase>V
      | %<VLF>pu
      | %<angleLF>deg.
      | %<Name>
  bus97 : powerlib/Measurements/Load Flow Bus  LConnTagsString=a  ID=bus97  Vbase=150000  Vref=1  Vangle=0  VLF=1  angleLF=0
      settings: AttributesFormatString=|
      | %<ID>
      | %<Vbase>V
      | %<VLF>pu
      | %<angleLF>deg.
      | %<Name>
  bus98 : powerlib/Measurements/Load Flow Bus  LConnTagsString=a  ID=bus98  Vbase=150000  Vref=1  Vangle=0  VLF=1  angleLF=0
      settings: AttributesFormatString=|
      | %<ID>
      | %<Vbase>V
      | %<VLF>pu
      | %<angleLF>deg.
      | %<Name>
  bus99 : powerlib/Measurements/Load Flow Bus  LConnTagsString=a  ID=bus99  Vbase=150000  Vref=1  Vangle=0  VLF=1  angleLF=0
      settings: AttributesFormatString=|
      | %<ID>
      | %<Vbase>V
      | %<VLF>pu
      | %<angleLF>deg.
      | %<Name>
  powergui : powerlib/powergui  Priority=1  SimulationMode=Continuous  SolverType=Tustin  SampleTime=50e-6  frequency=60  SPID=off  DisableSnubberDevices=off  DisableRonSwitches=off  DisableVfSwitches=off  SwTol=0  Interpol=off  DisplayEquations=off  Ts=0  methode=off  frequencyindice=60  Pbase=100e6  ErrMax=1e-4  Iterations=50  UnitsV=kV  UnitsW=MW  FunctionMessages=off  echomessages=off  HookPort=off  EnableUseOfTLC=off  x0status=blocks  RestoreLinks=warning  ResistiveCurrentMeasurement=off  Frange=[0:2:500]  Ylog=off  Xlog=on  ShowGrid=off  save=off  variable=ZData  structure=0  ZoomFFT=off  StartTime=0.0  cycles=1  DisplayStyle=1  fundamental=60  FreqAxis=off  MaxFrequency=1000  frequencyindicesteady=1  RmsSteady=1  display=off
  connections:
  _CN_268532907_150000_CN_268532908_150000/LConn1 -- T_268532907__/LConn1 -- _CN_268532907_150000_CN_399277121_150000/LConn1
  _CN_268532907_150000_CN_268532908_150000/LConn2 -- T_268532907__/LConn2 -- _CN_268532907_150000_CN_399277121_150000/LConn2
  _CN_268532907_150000_CN_268532908_150000/LConn3 -- T_268532907__/LConn3 -- _CN_268532907_150000_CN_399277121_150000/LConn3 -- bus1/LConn1
  T_268532908__/LConn1 -- _CN_268532907_150000_CN_268532908_150000/RConn1
  T_268532908__/LConn2 -- _CN_268532907_150000_CN_268532908_150000/RConn2
  _CN_268532907_150000_CN_268532908_150000/RConn3 -- T_268532908__/LConn3 -- bus2/LConn1
  _CN_268532907_150000_CN_399277121_150000/RConn1 -- T_399277121__/LConn1 -- _CN_268532906_150000_CN_399277121_150000/LConn1
  _CN_268532907_150000_CN_399277121_150000/RConn2 -- T_399277121__/LConn2 -- _CN_268532906_150000_CN_399277121_150000/LConn2
  _CN_268532907_150000_CN_399277121_150000/RConn3 -- T_399277121__/LConn3 -- _CN_268532906_150000_CN_399277121_150000/LConn3 -- bus3/LConn1
  _CN_261381125_150000_CN_264719089_150000/LConn1 -- T_261381125__/LConn1 -- _CN_261381125_150000_CN_166633831_150000/LConn1
  _CN_261381125_150000_CN_264719089_150000/LConn2 -- T_261381125__/LConn2 -- _CN_261381125_150000_CN_166633831_150000/LConn2
  _CN_261381125_150000_CN_264719089_150000/LConn3 -- T_261381125__/LConn3 -- _CN_261381125_150000_CN_166633831_150000/LConn3 -- bus4/LConn1
  _CN_261381125_150000_CN_264719089_150000/RConn1 -- T_264719089__/LConn1 -- _CN_264719089_150000_CN_261185003_150000/LConn1
  _CN_261381125_150000_CN_264719089_150000/RConn2 -- T_264719089__/LConn2 -- _CN_264719089_150000_CN_261185003_150000/LConn2
  _CN_261381125_150000_CN_264719089_150000/RConn3 -- T_264719089__/LConn3 -- _CN_264719089_150000_CN_261185003_150000/LConn3 -- bus5/LConn1
  _CN_261381125_150000_CN_166633831_150000/RConn1 -- T_166633831__/RConn1 -- _CN_166632018_150000_CN_166633831_150000/LConn1 -- _CN_104538467_150000_CN_166633831_150000/LConn1 -- L_166633831/LConn1
  _CN_261381125_150000_CN_166633831_150000/RConn2 -- T_166633831__/RConn2 -- _CN_166632018_150000_CN_166633831_150000/LConn2 -- _CN_104538467_150000_CN_166633831_150000/LConn2 -- L_166633831/LConn2
  _CN_261381125_150000_CN_166633831_150000/RConn3 -- T_166633831__/RConn3 -- _CN_166632018_150000_CN_166633831_150000/LConn3 -- _CN_104538467_150000_CN_166633831_150000/LConn3 -- L_166633831/LConn3 -- bus6/LConn1
  T_264072199__/LConn1 -- _CN_264072199_150000_CN_399057172_150000/LConn1
  T_264072199__/LConn2 -- _CN_264072199_150000_CN_399057172_150000/LConn2
  _CN_264072199_150000_CN_399057172_150000/LConn3 -- T_264072199__/LConn3 -- bus7/LConn1
  _CN_264072199_150000_CN_399057172_150000/RConn1 -- T_399057172__/LConn1 -- _CN_399057165_150000_CN_399057172_150000/LConn1 -- _CN_399057172_150000_CN_263932883_150000/LConn1
  _CN_264072199_150000_CN_399057172_150000/RConn2 -- T_399057172__/LConn2 -- _CN_399057165_150000_CN_399057172_150000/LConn2 -- _CN_399057172_150000_CN_263932883_150000/LConn2
  _CN_264072199_150000_CN_399057172_150000/RConn3 -- T_399057172__/LConn3 -- _CN_399057165_150000_CN_399057172_150000/LConn3 -- _CN_399057172_150000_CN_263932883_150000/LConn3 -- bus8/LConn1
  T_186634762__/LConn1 -- _CN_186634762_150000_CN_340152021_150000/LConn1
  T_186634762__/LConn2 -- _CN_186634762_150000_CN_340152021_150000/LConn2
  _CN_186634762_150000_CN_340152021_150000/LConn3 -- T_186634762__/LConn3 -- bus9/LConn1
  T_340152021__/LConn1 -- _CN_186634762_150000_CN_340152021_150000/RConn1
  T_340152021__/LConn2 -- _CN_186634762_150000_CN_340152021_150000/RConn2
  _CN_186634762_150000_CN_340152021_150000/RConn3 -- T_340152021__/LConn3 -- bus10/LConn1
  _CN_265318414_150000_CN_265318415_150000/LConn1 -- T_265318414__/RConn1 -- L_265318414/LConn1
  _CN_265318414_150000_CN_265318415_150000/LConn2 -- T_265318414__/RConn2 -- L_265318414/LConn2
  _CN_265318414_150000_CN_265318415_150000/LConn3 -- T_265318414__/RConn3 -- L_265318414/LConn3 -- bus11/LConn1
  _CN_265318414_150000_CN_265318415_150000/RConn1 -- T_265318415__/LConn1 -- _CN_265318415_150000_CN_268831422_150000/LConn1 -- _CN_268846126_150000_CN_265318415_150000/LConn1
  _CN_265318414_150000_CN_265318415_150000/RConn2 -- T_265318415__/LConn2 -- _CN_265318415_150000_CN_268831422_150000/LConn2 -- _CN_268846126_150000_CN_265318415_150000/LConn2
  _CN_265318414_150000_CN_265318415_150000/RConn3 -- T_265318415__/LConn3 -- _CN_265318415_150000_CN_268831422_150000/LConn3 -- bus12/LConn1 -- _CN_268846126_150000_CN_265318415_150000/LConn3
  T_246972431__/LConn1 -- _CN_246972431_150000_CN_234372891_150000/LConn1
  T_246972431__/LConn2 -- _CN_246972431_150000_CN_234372891_150000/LConn2
  _CN_246972431_150000_CN_234372891_150000/LConn3 -- T_246972431__/LConn3 -- bus13/LConn1
  T_234372891__/LConn1 -- _CN_246972431_150000_CN_234372891_150000/RConn1
  T_234372891__/LConn2 -- _CN_246972431_150000_CN_234372891_150000/RConn2
  _CN_246972431_150000_CN_234372891_150000/RConn3 -- T_234372891__/LConn3 -- bus14/LConn1
  T_269492241__/LConn1 -- _CN_269492241_150000_CN_269492237_150000/LConn1
  T_269492241__/LConn2 -- _CN_269492241_150000_CN_269492237_150000/LConn2
  _CN_269492241_150000_CN_269492237_150000/LConn3 -- T_269492241__/LConn3 -- bus15/LConn1
  _CN_269492241_150000_CN_269492237_150000/RConn1 -- G_269492237_Indramayu/RConn1 -- _CN_269475415_150000_CN_269492237_150000/LConn1
  _CN_269492241_150000_CN_269492237_150000/RConn2 -- G_269492237_Indramayu/RConn2 -- _CN_269475415_150000_CN_269492237_150000/LConn2
  _CN_269492241_150000_CN_269492237_150000/RConn3 -- G_269492237_Indramayu/RConn3 -- _CN_269475415_150000_CN_269492237_150000/LConn3 -- bus16/LConn1
  T_160831508__/LConn1 -- _CN_160831508_150000_CN_160831511_150000/LConn1
  T_160831508__/LConn2 -- _CN_160831508_150000_CN_160831511_150000/LConn2
  _CN_160831508_150000_CN_160831511_150000/LConn3 -- T_160831508__/LConn3 -- bus17/LConn1
  T_160831511__/LConn1 -- _CN_160831508_150000_CN_160831511_150000/RConn1
  T_160831511__/LConn2 -- _CN_160831508_150000_CN_160831511_150000/RConn2
  _CN_160831508_150000_CN_160831511_150000/RConn3 -- T_160831511__/LConn3 -- bus18/LConn1
  T_399067566__/LConn1 -- _CN_399067566_150000_CN_399067557_150000/LConn1
  T_399067566__/LConn2 -- _CN_399067566_150000_CN_399067557_150000/LConn2
  _CN_399067566_150000_CN_399067557_150000/LConn3 -- T_399067566__/LConn3 -- bus19/LConn1
  _CN_399067566_150000_CN_399067557_150000/RConn1 -- T_399067557__/LConn1 -- _CN_269475415_150000_CN_399067557_150000/LConn1
  _CN_399067566_150000_CN_399067557_150000/RConn2 -- T_399067557__/LConn2 -- _CN_269475415_150000_CN_399067557_150000/LConn2
  _CN_399067566_150000_CN_399067557_150000/RConn3 -- T_399067557__/LConn3 -- _CN_269475415_150000_CN_399067557_150000/LConn3 -- bus20/LConn1
  T_167008794__/LConn1 -- _CN_167008794_150000_CN_199476036_150000/LConn1
  T_167008794__/LConn2 -- _CN_167008794_150000_CN_199476036_150000/LConn2
  _CN_167008794_150000_CN_199476036_150000/LConn3 -- T_167008794__/LConn3 -- bus21/LConn1
  T_199476036__/LConn1 -- _CN_167008794_150000_CN_199476036_150000/RConn1
  T_199476036__/LConn2 -- _CN_167008794_150000_CN_199476036_150000/RConn2
  _CN_167008794_150000_CN_199476036_150000/RConn3 -- T_199476036__/LConn3 -- bus22/LConn1
  _CN_311479837_150000_CN_311980589_150000/LConn1 -- T_311479837__GITET_Gresik/RConn1 -- _CN_311479837_150000_CN_166644946_150000/LConn1 -- L_311479837/LConn1
  _CN_311479837_150000_CN_311980589_150000/LConn2 -- T_311479837__GITET_Gresik/RConn2 -- _CN_311479837_150000_CN_166644946_150000/LConn2 -- L_311479837/LConn2
  _CN_311479837_150000_CN_311980589_150000/LConn3 -- T_311479837__GITET_Gresik/RConn3 -- _CN_311479837_150000_CN_166644946_150000/LConn3 -- L_311479837/LConn3 -- bus23/LConn1
  T_311980589__Gardu_Induk_Alta_Prima/LConn1 -- _CN_311479837_150000_CN_311980589_150000/RConn1
  T_311980589__Gardu_Induk_Alta_Prima/LConn2 -- _CN_311479837_150000_CN_311980589_150000/RConn2
  _CN_311479837_150000_CN_311980589_150000/RConn3 -- T_311980589__Gardu_Induk_Alta_Prima/LConn3 -- bus24/LConn1
  _CN_311479837_150000_CN_166644946_150000/RConn1 -- T_166644946__Gardu_Induk_Surabaya_Barat/LConn1 -- _CN_166644946_150000_CN_311963427_150000/LConn1 -- _CN_166644946_150000_CN_311432988_150000/LConn1 -- _CN_166644946_150000_CN_340978671_150000/LConn1 -- _CN_166644946_150000_CN_311963425_150000/LConn1 -- _CN_311940754_150000_CN_166644946_150000/LConn1
  _CN_311479837_150000_CN_166644946_150000/RConn2 -- T_166644946__Gardu_Induk_Surabaya_Barat/LConn2 -- _CN_166644946_150000_CN_311963427_150000/LConn2 -- _CN_166644946_150000_CN_311432988_150000/LConn2 -- _CN_166644946_150000_CN_340978671_150000/LConn2 -- _CN_166644946_150000_CN_311963425_150000/LConn2 -- _CN_311940754_150000_CN_166644946_150000/LConn2
  _CN_311479837_150000_CN_166644946_150000/RConn3 -- T_166644946__Gardu_Induk_Surabaya_Barat/LConn3 -- _CN_166644946_150000_CN_311963427_150000/LConn3 -- bus25/LConn1 -- _CN_166644946_150000_CN_311432988_150000/LConn3 -- _CN_166644946_150000_CN_340978671_150000/LConn3 -- _CN_166644946_150000_CN_311963425_150000/LConn3 -- _CN_311940754_150000_CN_166644946_150000/LConn3
  T_277204741__/LConn1 -- _CN_277204741_150000_CN_276990481_150000/LConn1
  T_277204741__/LConn2 -- _CN_277204741_150000_CN_276990481_150000/LConn2
  _CN_277204741_150000_CN_276990481_150000/LConn3 -- T_277204741__/LConn3 -- bus26/LConn1
  _CN_277204741_150000_CN_276990481_150000/RConn1 -- T_276990481__/LConn1 -- _CN_276990481_150000_CN_277204263_150000/LConn1 -- _CN_276990481_150000_CN_340205049_150000/LConn1
  _CN_277204741_150000_CN_276990481_150000/RConn2 -- T_276990481__/LConn2 -- _CN_276990481_150000_CN_277204263_150000/LConn2 -- _CN_276990481_150000_CN_340205049_150000/LConn2
  _CN_277204741_150000_CN_276990481_150000/RConn3 -- T_276990481__/LConn3 -- _CN_276990481_150000_CN_277204263_150000/LConn3 -- _CN_276990481_150000_CN_340205049_150000/LConn3 -- bus27/LConn1
  _CN_228490272_150000_CN_265030543_150000/LConn1 -- T_228490272__Gardu_Induk_PLN_Palur/LConn1 -- _CN_228490272_150000_CN_268865917_150000/LConn1 -- _CN_228490272_150000_CN_104412357_150000/LConn1
  _CN_228490272_150000_CN_265030543_150000/LConn2 -- T_228490272__Gardu_Induk_PLN_Palur/LConn2 -- _CN_228490272_150000_CN_268865917_150000/LConn2 -- _CN_228490272_150000_CN_104412357_150000/LConn2
  _CN_228490272_150000_CN_265030543_150000/LConn3 -- T_228490272__Gardu_Induk_PLN_Palur/LConn3 -- _CN_228490272_150000_CN_268865917_150000/LConn3 -- _CN_228490272_150000_CN_104412357_150000/LConn3 -- bus28/LConn1
  _CN_228490272_150000_CN_265030543_150000/RConn1 -- T_265030543__/LConn1 -- _CN_104339545_150000_CN_265030543_150000/LConn1
  _CN_228490272_150000_CN_265030543_150000/RConn2 -- T_265030543__/LConn2 -- _CN_104339545_150000_CN_265030543_150000/LConn2
  _CN_228490272_150000_CN_265030543_150000/RConn3 -- T_265030543__/LConn3 -- _CN_104339545_150000_CN_265030543_150000/LConn3 -- bus29/LConn1
  _CN_228490272_150000_CN_268865917_150000/RConn1 -- T_268865917__/LConn1 -- _CN_268865913_150000_CN_268865917_150000/LConn1
  _CN_228490272_150000_CN_268865917_150000/RConn2 -- T_268865917__/LConn2 -- _CN_268865913_150000_CN_268865917_150000/LConn2
  _CN_228490272_150000_CN_268865917_150000/RConn3 -- T_268865917__/LConn3 -- _CN_268865913_150000_CN_268865917_150000/LConn3 -- bus30/LConn1
  _CN_228490272_150000_CN_104412357_150000/RConn1 -- T_104412357__/LConn1 -- _CN_104412357_150000_CN_104412331_150000/LConn1
  _CN_228490272_150000_CN_104412357_150000/RConn2 -- T_104412357__/LConn2 -- _CN_104412357_150000_CN_104412331_150000/LConn2
  _CN_228490272_150000_CN_104412357_150000/RConn3 -- T_104412357__/LConn3 -- _CN_104412357_150000_CN_104412331_150000/LConn3 -- bus31/LConn1
  _CN_311479841_150000_CN_311666431_150000/LConn1 -- T_311479841__Gardu_Sekar_Bungu/LConn1 -- _CN_311479841_150000_CN_311666430_150000/LConn1
  _CN_311479841_150000_CN_311666431_150000/LConn2 -- T_311479841__Gardu_Sekar_Bungu/LConn2 -- _CN_311479841_150000_CN_311666430_150000/LConn2
  _CN_311479841_150000_CN_311666431_150000/LConn3 -- T_311479841__Gardu_Sekar_Bungu/LConn3 -- _CN_311479841_150000_CN_311666430_150000/LConn3 -- bus32/LConn1
  T_311666431__Gardu_Induk_Gili_Timur/LConn1 -- _CN_311479841_150000_CN_311666431_150000/RConn1
  T_311666431__Gardu_Induk_Gili_Timur/LConn2 -- _CN_311479841_150000_CN_311666431_150000/RConn2
  _CN_311479841_150000_CN_311666431_150000/RConn3 -- T_311666431__Gardu_Induk_Gili_Timur/LConn3 -- bus33/LConn1
  _CN_311479841_150000_CN_311666430_150000/RConn1 -- T_311666430__Gardu_Induk_Bangkalan/LConn1 -- _CN_311666430_150000_CN_311666433_150000/LConn1
  _CN_311479841_150000_CN_311666430_150000/RConn2 -- T_311666430__Gardu_Induk_Bangkalan/LConn2 -- _CN_311666430_150000_CN_311666433_150000/LConn2
  _CN_311479841_150000_CN_311666430_150000/RConn3 -- T_311666430__Gardu_Induk_Bangkalan/LConn3 -- _CN_311666430_150000_CN_311666433_150000/LConn3 -- bus34/LConn1
  T_398909637__/LConn1 -- _CN_398909637_150000_CN_311485046_150000/LConn1
  T_398909637__/LConn2 -- _CN_398909637_150000_CN_311485046_150000/LConn2
  _CN_398909637_150000_CN_311485046_150000/LConn3 -- T_398909637__/LConn3 -- bus35/LConn1
  T_311485046__Gardu_Induk_Cerme/LConn1 -- _CN_398909637_150000_CN_311485046_150000/RConn1
  T_311485046__Gardu_Induk_Cerme/LConn2 -- _CN_398909637_150000_CN_311485046_150000/RConn2
  _CN_398909637_150000_CN_311485046_150000/RConn3 -- T_311485046__Gardu_Induk_Cerme/LConn3 -- bus36/LConn1
  _CN_264855643_150000_CN_265002737_150000/LConn1 -- T_264855643__/LConn1 -- _CN_264855643_150000_CN_271376029_150000/LConn1 -- _CN_264855643_150000_CN_264855645_150000/LConn1
  _CN_264855643_150000_CN_265002737_150000/LConn2 -- T_264855643__/LConn2 -- _CN_264855643_150000_CN_271376029_150000/LConn2 -- _CN_264855643_150000_CN_264855645_150000/LConn2
  _CN_264855643_150000_CN_265002737_150000/LConn3 -- T_264855643__/LConn3 -- _CN_264855643_150000_CN_271376029_150000/LConn3 -- bus37/LConn1 -- _CN_264855643_150000_CN_264855645_150000/LConn3
  T_265002737__/LConn1 -- _CN_264855643_150000_CN_265002737_150000/RConn1
  T_265002737__/LConn2 -- _CN_264855643_150000_CN_265002737_150000/RConn2
  _CN_264855643_150000_CN_265002737_150000/RConn3 -- T_265002737__/LConn3 -- bus38/LConn1
  _CN_264855643_150000_CN_264855645_150000/RConn1 -- T_264855645__/LConn1 -- _CN_264855645_150000_CN_399067568_150000/LConn1 -- _CN_264855645_150000_CN_237756221_150000/LConn1 -- _CN_264855645_150000_CN_264410228_150000/LConn1
  _CN_264855643_150000_CN_264855645_150000/RConn2 -- T_264855645__/LConn2 -- _CN_264855645_150000_CN_399067568_150000/LConn2 -- _CN_264855645_150000_CN_237756221_150000/LConn2 -- _CN_264855645_150000_CN_264410228_150000/LConn2
  _CN_264855643_150000_CN_264855645_150000/RConn3 -- T_264855645__/LConn3 -- _CN_264855645_150000_CN_399067568_150000/LConn3 -- _CN_264855645_150000_CN_237756221_150000/LConn3 -- _CN_264855645_150000_CN_264410228_150000/LConn3 -- bus39/LConn1
  G_271376029_/RConn1 -- _CN_264855643_150000_CN_271376029_150000/RConn1
  G_271376029_/RConn2 -- _CN_264855643_150000_CN_271376029_150000/RConn2
  _CN_264855643_150000_CN_271376029_150000/RConn3 -- G_271376029_/RConn3 -- bus40/LConn1
  T_248953893__/LConn1 -- _CN_248953893_150000_CN_248953894_150000/LConn1
  T_248953893__/LConn2 -- _CN_248953893_150000_CN_248953894_150000/LConn2
  _CN_248953893_150000_CN_248953894_150000/LConn3 -- T_248953893__/LConn3 -- bus41/LConn1
  T_248953894__/LConn1 -- _CN_248953893_150000_CN_248953894_150000/RConn1
  T_248953894__/LConn2 -- _CN_248953893_150000_CN_248953894_150000/RConn2
  _CN_248953893_150000_CN_248953894_150000/RConn3 -- T_248953894__/LConn3 -- bus42/LConn1
  T_267663602__/LConn1 -- _CN_267663602_150000_CN_279284589_150000/LConn1
  T_267663602__/LConn2 -- _CN_267663602_150000_CN_279284589_150000/LConn2
  _CN_267663602_150000_CN_279284589_150000/LConn3 -- T_267663602__/LConn3 -- bus43/LConn1
  _CN_267663602_150000_CN_279284589_150000/RConn1 -- T_279284589__/LConn1 -- _CN_265002738_150000_CN_279284589_150000/LConn1
  _CN_267663602_150000_CN_279284589_150000/RConn2 -- T_279284589__/LConn2 -- _CN_265002738_150000_CN_279284589_150000/LConn2
  _CN_267663602_150000_CN_279284589_150000/RConn3 -- T_279284589__/LConn3 -- _CN_265002738_150000_CN_279284589_150000/LConn3 -- bus44/LConn1
  _CN_195105324_150000_CN_398925619_150000/LConn1 -- T_195105324__/LConn1 -- _CN_195105324_150000_CN_195211467_150000/LConn1
  _CN_195105324_150000_CN_398925619_150000/LConn2 -- T_195105324__/LConn2 -- _CN_195105324_150000_CN_195211467_150000/LConn2
  _CN_195105324_150000_CN_398925619_150000/LConn3 -- T_195105324__/LConn3 -- _CN_195105324_150000_CN_195211467_150000/LConn3 -- bus45/LConn1
  _CN_195105324_150000_CN_398925619_150000/RConn1 -- T_398925619__/LConn1 -- _CN_265568004_150000_CN_398925619_150000/LConn1
  _CN_195105324_150000_CN_398925619_150000/RConn2 -- T_398925619__/LConn2 -- _CN_265568004_150000_CN_398925619_150000/LConn2
  _CN_195105324_150000_CN_398925619_150000/RConn3 -- T_398925619__/LConn3 -- _CN_265568004_150000_CN_398925619_150000/LConn3 -- bus46/LConn1
  T_195211467__/LConn1 -- _CN_195105324_150000_CN_195211467_150000/RConn1
  T_195211467__/LConn2 -- _CN_195105324_150000_CN_195211467_150000/RConn2
  _CN_195105324_150000_CN_195211467_150000/RConn3 -- T_195211467__/LConn3 -- bus47/LConn1
  _CN_268846126_150000_CN_268846115_150000/LConn1 -- T_268846126__/LConn1 -- _CN_268846126_150000_CN_265318415_150000/RConn1 -- _CN_268846126_150000_CN_268831411_150000/LConn1
  _CN_268846126_150000_CN_268846115_150000/LConn2 -- T_268846126__/LConn2 -- _CN_268846126_150000_CN_265318415_150000/RConn2 -- _CN_268846126_150000_CN_268831411_150000/LConn2
  _CN_268846126_150000_CN_268846115_150000/LConn3 -- T_268846126__/LConn3 -- _CN_268846126_150000_CN_265318415_150000/RConn3 -- _CN_268846126_150000_CN_268831411_150000/LConn3 -- bus48/LConn1
  T_268846115__/LConn1 -- _CN_268846126_150000_CN_268846115_150000/RConn1
  T_268846115__/LConn2 -- _CN_268846126_150000_CN_268846115_150000/RConn2
  _CN_268846126_150000_CN_268846115_150000/RConn3 -- T_268846115__/LConn3 -- bus49/LConn1
  _CN_268846126_150000_CN_268831411_150000/RConn1 -- T_268831411__/LConn1 -- _CN_268831411_150000_CN_268865913_150000/LConn1
  _CN_268846126_150000_CN_268831411_150000/RConn2 -- T_268831411__/LConn2 -- _CN_268831411_150000_CN_268865913_150000/LConn2
  _CN_268846126_150000_CN_268831411_150000/RConn3 -- T_268831411__/LConn3 -- _CN_268831411_150000_CN_268865913_150000/LConn3 -- bus50/LConn1
  _CN_399724591_150000_CN_257613250_150000/LConn1 -- T_399724591__/LConn1 -- _CN_399724591_150000_CN_399724593_150000/LConn1
  _CN_399724591_150000_CN_257613250_150000/LConn2 -- T_399724591__/LConn2 -- _CN_399724591_150000_CN_399724593_150000/LConn2
  _CN_399724591_150000_CN_257613250_150000/LConn3 -- T_399724591__/LConn3 -- _CN_399724591_150000_CN_399724593_150000/LConn3 -- bus51/LConn1
  G_257613250_/RConn1 -- _CN_399724591_150000_CN_257613250_150000/RConn1
  G_257613250_/RConn2 -- _CN_399724591_150000_CN_257613250_150000/RConn2
  _CN_399724591_150000_CN_257613250_150000/RConn3 -- G_257613250_/RConn3 -- bus52/LConn1
  T_399724593__/LConn1 -- _CN_399724591_150000_CN_399724593_150000/RConn1
  T_399724593__/LConn2 -- _CN_399724591_150000_CN_399724593_150000/RConn2
  _CN_399724591_150000_CN_399724593_150000/RConn3 -- T_399724593__/LConn3 -- bus53/LConn1
  _CN_162030133_150000_CN_162030143_150000/LConn1 -- T_162030133__/LConn1 -- _CN_162030133_150000_CN_263932883_150000/LConn1 -- _CN_162030133_150000_CN_162002076_150000/LConn1
  _CN_162030133_150000_CN_162030143_150000/LConn2 -- T_162030133__/LConn2 -- _CN_162030133_150000_CN_263932883_150000/LConn2 -- _CN_162030133_150000_CN_162002076_150000/LConn2
  _CN_162030133_150000_CN_162030143_150000/LConn3 -- T_162030133__/LConn3 -- _CN_162030133_150000_CN_263932883_150000/LConn3 -- bus54/LConn1 -- _CN_162030133_150000_CN_162002076_150000/LConn3
  T_162030143__/LConn1 -- _CN_162030133_150000_CN_162030143_150000/RConn1
  T_162030143__/LConn2 -- _CN_162030133_150000_CN_162030143_150000/RConn2
  _CN_162030133_150000_CN_162030143_150000/RConn3 -- T_162030143__/LConn3 -- bus55/LConn1
  _CN_162030133_150000_CN_162002076_150000/RConn1 -- T_162002076__/LConn1 -- _CN_161980511_150000_CN_162002076_150000/LConn1
  _CN_162030133_150000_CN_162002076_150000/RConn2 -- T_162002076__/LConn2 -- _CN_161980511_150000_CN_162002076_150000/LConn2
  _CN_162030133_150000_CN_162002076_150000/RConn3 -- T_162002076__/LConn3 -- _CN_161980511_150000_CN_162002076_150000/LConn3 -- bus56/LConn1
  _CN_162030133_150000_CN_263932883_150000/RConn1 -- T_263932883__/LConn1 -- _CN_399057172_150000_CN_263932883_150000/RConn1
  _CN_162030133_150000_CN_263932883_150000/RConn2 -- T_263932883__/LConn2 -- _CN_399057172_150000_CN_263932883_150000/RConn2
  _CN_162030133_150000_CN_263932883_150000/RConn3 -- T_263932883__/LConn3 -- _CN_399057172_150000_CN_263932883_150000/RConn3 -- bus57/LConn1
  _CN_311479840_150000_CN_311479839_150000/LConn1 -- T_311479840__Gardu_Induk_Segoromadu/LConn1 -- _CN_311479840_150000_CN_398909625_150000/LConn1
  _CN_311479840_150000_CN_311479839_150000/LConn2 -- T_311479840__Gardu_Induk_Segoromadu/LConn2 -- _CN_311479840_150000_CN_398909625_150000/LConn2
  _CN_311479840_150000_CN_311479839_150000/LConn3 -- T_311479840__Gardu_Induk_Segoromadu/LConn3 -- _CN_311479840_150000_CN_398909625_150000/LConn3 -- bus58/LConn1
  T_311479839__Gardu_Induk_Petrokimia/LConn1 -- _CN_311479840_150000_CN_311479839_150000/RConn1
  T_311479839__Gardu_Induk_Petrokimia/LConn2 -- _CN_311479840_150000_CN_311479839_150000/RConn2
  _CN_311479840_150000_CN_311479839_150000/RConn3 -- T_311479839__Gardu_Induk_Petrokimia/LConn3 -- bus59/LConn1
  T_398909625__/LConn1 -- _CN_311479840_150000_CN_398909625_150000/RConn1
  T_398909625__/LConn2 -- _CN_311479840_150000_CN_398909625_150000/RConn2
  _CN_311479840_150000_CN_398909625_150000/RConn3 -- T_398909625__/LConn3 -- bus60/LConn1
  _CN_161951304_150000_CN_399038176_150000/LConn1 -- T_161951304__/LConn1 -- _CN_161951304_150000_CN_399038175_150000/LConn1 -- _CN_161951304_150000_CN_161948635_150000/LConn1
  _CN_161951304_150000_CN_399038176_150000/LConn2 -- T_161951304__/LConn2 -- _CN_161951304_150000_CN_399038175_150000/LConn2 -- _CN_161951304_150000_CN_161948635_150000/LConn2
  _CN_161951304_150000_CN_399038176_150000/LConn3 -- T_161951304__/LConn3 -- _CN_161951304_150000_CN_399038175_150000/LConn3 -- _CN_161951304_150000_CN_161948635_150000/LConn3 -- bus61/LConn1
  T_399038176__/LConn1 -- _CN_161951304_150000_CN_399038176_150000/RConn1
  T_399038176__/LConn2 -- _CN_161951304_150000_CN_399038176_150000/RConn2
  _CN_161951304_150000_CN_399038176_150000/RConn3 -- T_399038176__/LConn3 -- bus62/LConn1
  T_399038175__/LConn1 -- _CN_161951304_150000_CN_399038175_150000/RConn1
  T_399038175__/LConn2 -- _CN_161951304_150000_CN_399038175_150000/RConn2
  _CN_161951304_150000_CN_399038175_150000/RConn3 -- T_399038175__/LConn3 -- bus63/LConn1
  _CN_161951304_150000_CN_161948635_150000/RConn1 -- T_161948635__/LConn1 -- _CN_161948309_150000_CN_161948635_150000/LConn1
  _CN_161951304_150000_CN_161948635_150000/RConn2 -- T_161948635__/LConn2 -- _CN_161948309_150000_CN_161948635_150000/LConn2
  _CN_161951304_150000_CN_161948635_150000/RConn3 -- T_161948635__/LConn3 -- _CN_161948309_150000_CN_161948635_150000/LConn3 -- bus64/LConn1
  _CN_264713291_150000_CN_264713279_150000/LConn1 -- T_264713291__/RConn1 -- L_264713291/LConn1
  _CN_264713291_150000_CN_264713279_150000/LConn2 -- T_264713291__/RConn2 -- L_264713291/LConn2
  _CN_264713291_150000_CN_264713279_150000/LConn3 -- T_264713291__/RConn3 -- L_264713291/LConn3 -- bus65/LConn1
  _CN_264713291_150000_CN_264713279_150000/RConn1 -- T_264713279__/LConn1 -- _CN_264713279_150000_CN_153303534_150000/LConn1
  _CN_264713291_150000_CN_264713279_150000/RConn2 -- T_264713279__/LConn2 -- _CN_264713279_150000_CN_153303534_150000/LConn2
  _CN_264713291_150000_CN_264713279_150000/RConn3 -- T_264713279__/LConn3 -- _CN_264713279_150000_CN_153303534_150000/LConn3 -- bus66/LConn1
  _CN_269129296_150000_CN_399067568_150000/LConn1 -- T_269129296__/LConn1 -- _CN_269129296_150000_CN_265923575_150000/LConn1 -- _CN_269129296_150000_CN_261185002_150000/LConn1 -- _CN_269129296_150000_CN_269468436_150000/LConn1
  _CN_269129296_150000_CN_399067568_150000/LConn2 -- T_269129296__/LConn2 -- _CN_269129296_150000_CN_265923575_150000/LConn2 -- _CN_269129296_150000_CN_261185002_150000/LConn2 -- _CN_269129296_150000_CN_269468436_150000/LConn2
  _CN_269129296_150000_CN_399067568_150000/LConn3 -- T_269129296__/LConn3 -- _CN_269129296_150000_CN_265923575_150000/LConn3 -- _CN_269129296_150000_CN_261185002_150000/LConn3 -- _CN_269129296_150000_CN_269468436_150000/LConn3 -- bus67/LConn1
  _CN_269129296_150000_CN_399067568_150000/RConn1 -- T_399067568__/LConn1 -- _CN_264855645_150000_CN_399067568_150000/RConn1
  _CN_269129296_150000_CN_399067568_150000/RConn2 -- T_399067568__/LConn2 -- _CN_264855645_150000_CN_399067568_150000/RConn2
  _CN_269129296_150000_CN_399067568_150000/RConn3 -- T_399067568__/LConn3 -- _CN_264855645_150000_CN_399067568_150000/RConn3 -- bus68/LConn1
  _CN_269129296_150000_CN_265923575_150000/RConn1 -- T_265923575__/LConn1 -- _CN_166699717_150000_CN_265923575_150000/LConn1
  _CN_269129296_150000_CN_265923575_150000/RConn2 -- T_265923575__/LConn2 -- _CN_166699717_150000_CN_265923575_150000/LConn2
  _CN_269129296_150000_CN_265923575_150000/RConn3 -- T_265923575__/LConn3 -- _CN_166699717_150000_CN_265923575_150000/LConn3 -- bus69/LConn1
  _CN_269129296_150000_CN_261185002_150000/RConn1 -- T_261185002__/RConn1 -- L_261185002/LConn1
  _CN_269129296_150000_CN_261185002_150000/RConn2 -- T_261185002__/RConn2 -- L_261185002/LConn2
  _CN_269129296_150000_CN_261185002_150000/RConn3 -- T_261185002__/RConn3 -- L_261185002/LConn3 -- bus70/LConn1
  _CN_269129296_150000_CN_269468436_150000/RConn1 -- T_269468436__Gardu_Induk_PT__PLN/LConn1 -- _CN_269468436_150000_CN_271678852_150000/LConn1
  _CN_269129296_150000_CN_269468436_150000/RConn2 -- T_269468436__Gardu_Induk_PT__PLN/LConn2 -- _CN_269468436_150000_CN_271678852_150000/LConn2
  _CN_269129296_150000_CN_269468436_150000/RConn3 -- T_269468436__Gardu_Induk_PT__PLN/LConn3 -- _CN_269468436_150000_CN_271678852_150000/LConn3 -- bus71/LConn1
  _CN_166632018_150000_CN_104440761_150000/LConn1 -- T_166632018__/LConn1 -- _CN_166632018_150000_CN_270800486_150000/LConn1 -- _CN_166632018_150000_CN_265568004_150000/LConn1 -- _CN_166632018_150000_CN_104538467_150000/LConn1 -- _CN_166632018_150000_CN_166633831_150000/RConn1
  _CN_166632018_150000_CN_104440761_150000/LConn2 -- T_166632018__/LConn2 -- _CN_166632018_150000_CN_270800486_150000/LConn2 -- _CN_166632018_150000_CN_265568004_150000/LConn2 -- _CN_166632018_150000_CN_104538467_150000/LConn2 -- _CN_166632018_150000_CN_166633831_150000/RConn2
  _CN_166632018_150000_CN_104440761_150000/LConn3 -- T_166632018__/LConn3 -- _CN_166632018_150000_CN_270800486_150000/LConn3 -- _CN_166632018_150000_CN_265568004_150000/LConn3 -- _CN_166632018_150000_CN_104538467_150000/LConn3 -- _CN_166632018_150000_CN_166633831_150000/RConn3 -- bus72/LConn1
  _CN_166632018_150000_CN_104440761_150000/RConn1 -- T_104440761__/LConn1 -- _CN_104440761_150000_CN_265588689_150000/LConn1
  _CN_166632018_150000_CN_104440761_150000/RConn2 -- T_104440761__/LConn2 -- _CN_104440761_150000_CN_265588689_150000/LConn2
  _CN_166632018_150000_CN_104440761_150000/RConn3 -- T_104440761__/LConn3 -- _CN_104440761_150000_CN_265588689_150000/LConn3 -- bus73/LConn1
  T_270800486__/LConn1 -- _CN_166632018_150000_CN_270800486_150000/RConn1
  T_270800486__/LConn2 -- _CN_166632018_150000_CN_270800486_150000/RConn2
  _CN_166632018_150000_CN_270800486_150000/RConn3 -- T_270800486__/LConn3 -- bus74/LConn1
  _CN_166632018_150000_CN_265568004_150000/RConn1 -- T_265568004__/LConn1 -- _CN_265568004_150000_CN_398925619_150000/RConn1
  _CN_166632018_150000_CN_265568004_150000/RConn2 -- T_265568004__/LConn2 -- _CN_265568004_150000_CN_398925619_150000/RConn2
  _CN_166632018_150000_CN_265568004_150000/RConn3 -- T_265568004__/LConn3 -- _CN_265568004_150000_CN_398925619_150000/RConn3 -- bus75/LConn1
  _CN_166632018_150000_CN_104538467_150000/RConn1 -- T_104538467__/LConn1 -- _CN_104538467_150000_CN_166633831_150000/RConn1
  _CN_166632018_150000_CN_104538467_150000/RConn2 -- T_104538467__/LConn2 -- _CN_104538467_150000_CN_166633831_150000/RConn2
  _CN_166632018_150000_CN_104538467_150000/RConn3 -- T_104538467__/LConn3 -- _CN_104538467_150000_CN_166633831_150000/RConn3 -- bus76/LConn1
  _CN_269475415_150000_CN_399067557_150000/RConn1 -- T_269475415__/LConn1 -- _CN_269475415_150000_CN_269490141_150000/LConn1 -- _CN_269475415_150000_CN_269490147_150000/LConn1 -- _CN_269475415_150000_CN_269492237_150000/RConn1 -- _CN_269475415_150000_CN_399067565_150000/LConn1
  _CN_269475415_150000_CN_399067557_150000/RConn2 -- T_269475415__/LConn2 -- _CN_269475415_150000_CN_269490141_150000/LConn2 -- _CN_269475415_150000_CN_269490147_150000/LConn2 -- _CN_269475415_150000_CN_269492237_150000/RConn2 -- _CN_269475415_150000_CN_399067565_150000/LConn2
  _CN_269475415_150000_CN_399067557_150000/RConn3 -- T_269475415__/LConn3 -- _CN_269475415_150000_CN_269490141_150000/LConn3 -- _CN_269475415_150000_CN_269490147_150000/LConn3 -- bus77/LConn1 -- _CN_269475415_150000_CN_269492237_150000/RConn3 -- _CN_269475415_150000_CN_399067565_150000/LConn3
  T_399067565__/LConn1 -- _CN_269475415_150000_CN_399067565_150000/RConn1
  T_399067565__/LConn2 -- _CN_269475415_150000_CN_399067565_150000/RConn2
  _CN_269475415_150000_CN_399067565_150000/RConn3 -- T_399067565__/LConn3 -- bus78/LConn1
  T_269490141__/LConn1 -- _CN_269475415_150000_CN_269490141_150000/RConn1
  T_269490141__/LConn2 -- _CN_269475415_150000_CN_269490141_150000/RConn2
  _CN_269475415_150000_CN_269490141_150000/RConn3 -- T_269490141__/LConn3 -- bus79/LConn1
  _CN_269475415_150000_CN_269490147_150000/RConn1 -- T_269490147__/LConn1 -- _CN_269490135_150000_CN_269490147_150000/LConn1
  _CN_269475415_150000_CN_269490147_150000/RConn2 -- T_269490147__/LConn2 -- _CN_269490135_150000_CN_269490147_150000/LConn2
  _CN_269475415_150000_CN_269490147_150000/RConn3 -- T_269490147__/LConn3 -- _CN_269490135_150000_CN_269490147_150000/LConn3 -- bus80/LConn1
  T_269129304__/LConn1 -- _CN_269129304_150000_CN_264410228_150000/LConn1
  T_269129304__/LConn2 -- _CN_269129304_150000_CN_264410228_150000/LConn2
  _CN_269129304_150000_CN_264410228_150000/LConn3 -- T_269129304__/LConn3 -- bus81/LConn1
  _CN_269129304_150000_CN_264410228_150000/RConn1 -- T_264410228__/LConn1 -- _CN_264855645_150000_CN_264410228_150000/RConn1 -- _CN_264410228_150000_CN_269129291_150000/LConn1
  _CN_269129304_150000_CN_264410228_150000/RConn2 -- T_264410228__/LConn2 -- _CN_264855645_150000_CN_264410228_150000/RConn2 -- _CN_264410228_150000_CN_269129291_150000/LConn2
  _CN_269129304_150000_CN_264410228_150000/RConn3 -- T_264410228__/LConn3 -- _CN_264855645_150000_CN_264410228_150000/RConn3 -- _CN_264410228_150000_CN_269129291_150000/LConn3 -- bus82/LConn1
  _CN_104339545_150000_CN_265903214_150000/LConn1 -- T_104339545__/RConn1 -- _CN_104339545_150000_CN_265030543_150000/RConn1 -- _CN_104339545_150000_CN_104412331_150000/LConn1 -- _CN_104339545_150000_CN_265903215_150000/LConn1 -- _CN_104339545_150000_CN_265588689_150000/LConn1 -- _CN_104339545_150000_CN_121677176_150000/LConn1 -- L_104339545/LConn1
  _CN_104339545_150000_CN_265903214_150000/LConn2 -- T_104339545__/RConn2 -- _CN_104339545_150000_CN_265030543_150000/RConn2 -- _CN_104339545_150000_CN_104412331_150000/LConn2 -- _CN_104339545_150000_CN_265903215_150000/LConn2 -- _CN_104339545_150000_CN_265588689_150000/LConn2 -- _CN_104339545_150000_CN_121677176_150000/LConn2 -- L_104339545/LConn2
  _CN_104339545_150000_CN_265903214_150000/LConn3 -- T_104339545__/RConn3 -- _CN_104339545_150000_CN_265030543_150000/RConn3 -- _CN_104339545_150000_CN_104412331_150000/LConn3 -- _CN_104339545_150000_CN_265903215_150000/LConn3 -- _CN_104339545_150000_CN_265588689_150000/LConn3 -- _CN_104339545_150000_CN_121677176_150000/LConn3 -- L_104339545/LConn3 -- bus83/LConn1
  _CN_104339545_150000_CN_265903214_150000/RConn1 -- T_265903214__/LConn1 -- _CN_265903200_150000_CN_265903214_150000/LConn1
  _CN_104339545_150000_CN_265903214_150000/RConn2 -- T_265903214__/LConn2 -- _CN_265903200_150000_CN_265903214_150000/LConn2
  _CN_104339545_150000_CN_265903214_150000/RConn3 -- T_265903214__/LConn3 -- _CN_265903200_150000_CN_265903214_150000/LConn3 -- bus84/LConn1
  _CN_104339545_150000_CN_104412331_150000/RConn1 -- T_104412331__/LConn1 -- _CN_104412357_150000_CN_104412331_150000/RConn1 -- _CN_104412331_150000_CN_265030533_150000/LConn1
  _CN_104339545_150000_CN_104412331_150000/RConn2 -- T_104412331__/LConn2 -- _CN_104412357_150000_CN_104412331_150000/RConn2 -- _CN_104412331_150000_CN_265030533_150000/LConn2
  _CN_104339545_150000_CN_104412331_150000/RConn3 -- T_104412331__/LConn3 -- _CN_104412357_150000_CN_104412331_150000/RConn3 -- _CN_104412331_150000_CN_265030533_150000/LConn3 -- bus85/LConn1
  _CN_104339545_150000_CN_265903215_150000/RConn1 -- T_265903215__/LConn1 -- _CN_265903215_150000_CN_268532906_150000/LConn1
  _CN_104339545_150000_CN_265903215_150000/RConn2 -- T_265903215__/LConn2 -- _CN_265903215_150000_CN_268532906_150000/LConn2
  _CN_104339545_150000_CN_265903215_150000/RConn3 -- T_265903215__/LConn3 -- _CN_265903215_150000_CN_268532906_150000/LConn3 -- bus86/LConn1
  _CN_104339545_150000_CN_265588689_150000/RConn1 -- T_265588689__/LConn1 -- _CN_104440761_150000_CN_265588689_150000/RConn1
  _CN_104339545_150000_CN_265588689_150000/RConn2 -- T_265588689__/LConn2 -- _CN_104440761_150000_CN_265588689_150000/RConn2
  _CN_104339545_150000_CN_265588689_150000/RConn3 -- T_265588689__/LConn3 -- _CN_104440761_150000_CN_265588689_150000/RConn3 -- bus87/LConn1
  T_121677176__Gardu_PLN_150KV_Banteng/LConn1 -- _CN_104339545_150000_CN_121677176_150000/RConn1
  T_121677176__Gardu_PLN_150KV_Banteng/LConn2 -- _CN_104339545_150000_CN_121677176_150000/RConn2
  _CN_104339545_150000_CN_121677176_150000/RConn3 -- T_121677176__Gardu_PLN_150KV_Banteng/LConn3 -- bus88/LConn1
  T_399022980__/LConn1 -- _CN_399022980_150000_CN_271376043_150000/LConn1
  T_399022980__/LConn2 -- _CN_399022980_150000_CN_271376043_150000/LConn2
  _CN_399022980_150000_CN_271376043_150000/LConn3 -- T_399022980__/LConn3 -- bus89/LConn1
  _CN_399022980_150000_CN_271376043_150000/RConn1 -- T_271376043__/LConn1 -- _CN_271376043_150000_CN_269508907_150000/LConn1 -- _CN_271376043_150000_CN_153303534_150000/LConn1
  _CN_399022980_150000_CN_271376043_150000/RConn2 -- T_271376043__/LConn2 -- _CN_271376043_150000_CN_269508907_150000/LConn2 -- _CN_271376043_150000_CN_153303534_150000/LConn2
  _CN_399022980_150000_CN_271376043_150000/RConn3 -- T_271376043__/LConn3 -- _CN_271376043_150000_CN_269508907_150000/LConn3 -- _CN_271376043_150000_CN_153303534_150000/LConn3 -- bus90/LConn1
  T_268831422__/LConn1 -- _CN_265318415_150000_CN_268831422_150000/RConn1
  T_268831422__/LConn2 -- _CN_265318415_150000_CN_268831422_150000/RConn2
  _CN_265318415_150000_CN_268831422_150000/RConn3 -- T_268831422__/LConn3 -- bus91/LConn1
  G_237756221_PT__Star_Energy_Geothermal/RConn1 -- _CN_264855645_150000_CN_237756221_150000/RConn1
  G_237756221_PT__Star_Energy_Geothermal/RConn2 -- _CN_264855645_150000_CN_237756221_150000/RConn2
  _CN_264855645_150000_CN_237756221_150000/RConn3 -- G_237756221_PT__Star_Energy_Geothermal/RConn3 -- bus92/LConn1
  _CN_161980511_150000_CN_162002076_150000/RConn1 -- T_161980511__/LConn1 -- _CN_161980511_150000_CN_161980518_150000/LConn1
  _CN_161980511_150000_CN_162002076_150000/RConn2 -- T_161980511__/LConn2 -- _CN_161980511_150000_CN_161980518_150000/LConn2
  _CN_161980511_150000_CN_162002076_150000/RConn3 -- T_161980511__/LConn3 -- _CN_161980511_150000_CN_161980518_150000/LConn3 -- bus93/LConn1
  T_161980518__/LConn1 -- _CN_161980511_150000_CN_161980518_150000/RConn1
  T_161980518__/LConn2 -- _CN_161980511_150000_CN_161980518_150000/RConn2
  _CN_161980511_150000_CN_161980518_150000/RConn3 -- T_161980518__/LConn3 -- bus94/LConn1
  T_265903200__/LConn1 -- _CN_265903200_150000_CN_265903214_150000/RConn1
  T_265903200__/LConn2 -- _CN_265903200_150000_CN_265903214_150000/RConn2
  _CN_265903200_150000_CN_265903214_150000/RConn3 -- T_265903200__/LConn3 -- bus95/LConn1
  _CN_276990481_150000_CN_277204263_150000/RConn1 -- T_277204263__/LConn1 -- _CN_277204263_150000_CN_277204262_150000/LConn1 -- _CN_277204263_150000_CN_277183760_150000/LConn1
  _CN_276990481_150000_CN_277204263_150000/RConn2 -- T_277204263__/LConn2 -- _CN_277204263_150000_CN_277204262_150000/LConn2 -- _CN_277204263_150000_CN_277183760_150000/LConn2
  _CN_276990481_150000_CN_277204263_150000/RConn3 -- T_277204263__/LConn3 -- _CN_277204263_150000_CN_277204262_150000/LConn3 -- _CN_277204263_150000_CN_277183760_150000/LConn3 -- bus96/LConn1
  _CN_276990481_150000_CN_340205049_150000/RConn1 -- T_340205049__/LConn1 -- _CN_277183761_150000_CN_340205049_150000/LConn1
  _CN_276990481_150000_CN_340205049_150000/RConn2 -- T_340205049__/LConn2 -- _CN_277183761_150000_CN_340205049_150000/LConn2
  _CN_276990481_150000_CN_340205049_150000/RConn3 -- T_340205049__/LConn3 -- _CN_277183761_150000_CN_340205049_150000/LConn3 -- bus97/LConn1
  _CN_265903215_150000_CN_268532906_150000/RConn1 -- T_268532906__/LConn1 -- _CN_268532906_150000_CN_399277121_150000/RConn1
  _CN_265903215_150000_CN_268532906_150000/RConn2 -- T_268532906__/LConn2 -- _CN_268532906_150000_CN_399277121_150000/RConn2
  _CN_265903215_150000_CN_268532906_150000/RConn3 -- T_268532906__/LConn3 -- _CN_268532906_150000_CN_399277121_150000/RConn3 -- bus98/LConn1
  _CN_264410228_150000_CN_269129291_150000/RConn1 -- T_269129291__/LConn1 -- _CN_269129291_150000_CN_272989134_150000/LConn1 -- _CN_269129291_150000_CN_399094735_150000/LConn1
  _CN_264410228_150000_CN_269129291_150000/RConn2 -- T_269129291__/LConn2 -- _CN_269129291_150000_CN_272989134_150000/LConn2 -- _CN_269129291_150000_CN_399094735_150000/LConn2
  _CN_264410228_150000_CN_269129291_150000/RConn3 -- T_269129291__/LConn3 -- _CN_269129291_150000_CN_272989134_150000/LConn3 -- _CN_269129291_150000_CN_399094735_150000/LConn3 -- bus99/LConn1
  T_339802233__/LConn1 -- _CN_339802233_150000_CN_192989828_150000/LConn1
  T_339802233__/LConn2 -- _CN_339802233_150000_CN_192989828_150000/LConn2
  _CN_339802233_150000_CN_192989828_150000/LConn3 -- T_339802233__/LConn3 -- bus100/LConn1
  _CN_339802233_150000_CN_192989828_150000/RConn1 -- T_192989828__/LConn1 -- _CN_192989828_150000_CN_339792684_150000/LConn1 -- _CN_192989828_150000_CN_339796954_150000/LConn1
  _CN_339802233_150000_CN_192989828_150000/RConn2 -- T_192989828__/LConn2 -- _CN_192989828_150000_CN_339792684_150000/LConn2 -- _CN_192989828_150000_CN_339796954_150000/LConn2
  _CN_339802233_150000_CN_192989828_150000/RConn3 -- T_192989828__/LConn3 -- _CN_192989828_150000_CN_339792684_150000/LConn3 -- _CN_192989828_150000_CN_339796954_150000/LConn3 -- bus101/LConn1
  _CN_192989828_150000_CN_339792684_150000/RConn1 -- T_339792684__/LConn1 -- _CN_339792673_150000_CN_339792684_150000/LConn1 -- _CN_339792684_150000_CN_339792680_150000/LConn1 -- _CN_339792684_150000_CN_185683916_150000/LConn1 -- _CN_339792684_150000_CN_339792685_150000/LConn1
  _CN_192989828_150000_CN_339792684_150000/RConn2 -- T_339792684__/LConn2 -- _CN_339792673_150000_CN_339792684_150000/LConn2 -- _CN_339792684_150000_CN_339792680_150000/LConn2 -- _CN_339792684_150000_CN_185683916_150000/LConn2 -- _CN_339792684_150000_CN_339792685_150000/LConn2
  _CN_192989828_150000_CN_339792684_150000/RConn3 -- T_339792684__/LConn3 -- _CN_339792673_150000_CN_339792684_150000/LConn3 -- _CN_339792684_150000_CN_339792680_150000/LConn3 -- _CN_339792684_150000_CN_185683916_150000/LConn3 -- _CN_339792684_150000_CN_339792685_150000/LConn3 -- bus102/LConn1
  T_339796954__/LConn1 -- _CN_192989828_150000_CN_339796954_150000/RConn1
  T_339796954__/LConn2 -- _CN_192989828_150000_CN_339796954_150000/RConn2
  _CN_192989828_150000_CN_339796954_150000/RConn3 -- T_339796954__/LConn3 -- bus103/LConn1
  T_340935922__/LConn1 -- _CN_340935922_150000_CN_340963798_150000/LConn1
  T_340935922__/LConn2 -- _CN_340935922_150000_CN_340963798_150000/LConn2
  _CN_340935922_150000_CN_340963798_150000/LConn3 -- T_340935922__/LConn3 -- bus104/LConn1
  _CN_340935922_150000_CN_340963798_150000/RConn1 -- T_340963798__/LConn1 -- _CN_340963798_150000_CN_340947951_150000/LConn1 -- _CN_299352934_150000_CN_340963798_150000/LConn1
  _CN_340935922_150000_CN_340963798_150000/RConn2 -- T_340963798__/LConn2 -- _CN_340963798_150000_CN_340947951_150000/LConn2 -- _CN_299352934_150000_CN_340963798_150000/LConn2
  _CN_340935922_150000_CN_340963798_150000/RConn3 -- T_340963798__/LConn3 -- _CN_340963798_150000_CN_340947951_150000/LConn3 -- bus105/LConn1 -- _CN_299352934_150000_CN_340963798_150000/LConn3
  _CN_311940754_150000_CN_311942142_150000/LConn1 -- T_311940754__Gardu_Induk_Krembangan/LConn1 -- _CN_311940754_150000_CN_265568001_150000/LConn1 -- _CN_311940754_150000_CN_166644946_150000/RConn1
  _CN_311940754_150000_CN_311942142_150000/LConn2 -- T_311940754__Gardu_Induk_Krembangan/LConn2 -- _CN_311940754_150000_CN_265568001_150000/LConn2 -- _CN_311940754_150000_CN_166644946_150000/RConn2
  _CN_311940754_150000_CN_311942142_150000/LConn3 -- T_311940754__Gardu_Induk_Krembangan/LConn3 -- _CN_311940754_150000_CN_265568001_150000/LConn3 -- _CN_311940754_150000_CN_166644946_150000/RConn3 -- bus106/LConn1
  T_311942142__Gardu_Induk_Tandes/LConn1 -- _CN_311940754_150000_CN_311942142_150000/RConn1
  T_311942142__Gardu_Induk_Tandes/LConn2 -- _CN_311940754_150000_CN_311942142_150000/RConn2
  _CN_311940754_150000_CN_311942142_150000/RConn3 -- T_311942142__Gardu_Induk_Tandes/LConn3 -- bus107/LConn1
  _CN_311940754_150000_CN_265568001_150000/RConn1 -- T_265568001__GITET_Krian/RConn1 -- L_265568001/LConn1
  _CN_311940754_150000_CN_265568001_150000/RConn2 -- T_265568001__GITET_Krian/RConn2 -- L_265568001/LConn2
  _CN_311940754_150000_CN_265568001_150000/RConn3 -- T_265568001__GITET_Krian/RConn3 -- L_265568001/LConn3 -- bus108/LConn1
  T_267968147__/LConn1 -- _CN_267968147_150000_CN_269160480_150000/LConn1
  T_267968147__/LConn2 -- _CN_267968147_150000_CN_269160480_150000/LConn2
  _CN_267968147_150000_CN_269160480_150000/LConn3 -- T_267968147__/LConn3 -- bus109/LConn1
  _CN_267968147_150000_CN_269160480_150000/RConn1 -- T_269160480__/LConn1 -- _CN_269160480_150000_CN_261184996_150000/LConn1
  _CN_267968147_150000_CN_269160480_150000/RConn2 -- T_269160480__/LConn2 -- _CN_269160480_150000_CN_261184996_150000/LConn2
  _CN_267968147_150000_CN_269160480_150000/RConn3 -- T_269160480__/LConn3 -- _CN_269160480_150000_CN_261184996_150000/LConn3 -- bus110/LConn1
  _CN_161948309_150000_CN_161948635_150000/RConn1 -- T_161948309__/LConn1 -- _CN_161948309_150000_CN_161948315_150000/LConn1
  _CN_161948309_150000_CN_161948635_150000/RConn2 -- T_161948309__/LConn2 -- _CN_161948309_150000_CN_161948315_150000/LConn2
  _CN_161948309_150000_CN_161948635_150000/RConn3 -- T_161948309__/LConn3 -- _CN_161948309_150000_CN_161948315_150000/LConn3 -- bus111/LConn1
  _CN_161948309_150000_CN_161948315_150000/RConn1 -- T_161948315__/LConn1 -- _CN_161948315_150000_CN_399038178_150000/LConn1 -- _CN_161948315_150000_CN_399038179_150000/LConn1
  _CN_161948309_150000_CN_161948315_150000/RConn2 -- T_161948315__/LConn2 -- _CN_161948315_150000_CN_399038178_150000/LConn2 -- _CN_161948315_150000_CN_399038179_150000/LConn2
  _CN_161948309_150000_CN_161948315_150000/RConn3 -- T_161948315__/LConn3 -- _CN_161948315_150000_CN_399038178_150000/LConn3 -- _CN_161948315_150000_CN_399038179_150000/LConn3 -- bus112/LConn1
  _CN_116023446_150000_CN_229039262_150000/LConn1 -- T_116023446__/LConn1 -- _CN_116023446_150000_CN_116023450_150000/LConn1
  _CN_116023446_150000_CN_229039262_150000/LConn2 -- T_116023446__/LConn2 -- _CN_116023446_150000_CN_116023450_150000/LConn2
  _CN_116023446_150000_CN_229039262_150000/LConn3 -- T_116023446__/LConn3 -- _CN_116023446_150000_CN_116023450_150000/LConn3 -- bus113/LConn1
  T_229039262__/LConn1 -- _CN_116023446_150000_CN_229039262_150000/RConn1
  T_229039262__/LConn2 -- _CN_116023446_150000_CN_229039262_150000/RConn2
  _CN_116023446_150000_CN_229039262_150000/RConn3 -- T_229039262__/LConn3 -- bus114/LConn1
  _CN_116023446_150000_CN_116023450_150000/RConn1 -- T_116023450__/LConn1 -- _CN_116023450_150000_CN_109924603_150000/LConn1 -- _CN_116023450_150000_CN_399505626_150000/LConn1 -- _CN_116023450_150000_CN_399505633_150000/LConn1
  _CN_116023446_150000_CN_116023450_150000/RConn2 -- T_116023450__/LConn2 -- _CN_116023450_150000_CN_109924603_150000/LConn2 -- _CN_116023450_150000_CN_399505626_150000/LConn2 -- _CN_116023450_150000_CN_399505633_150000/LConn2
  _CN_116023446_150000_CN_116023450_150000/RConn3 -- T_116023450__/LConn3 -- _CN_116023450_150000_CN_109924603_150000/LConn3 -- _CN_116023450_150000_CN_399505626_150000/LConn3 -- _CN_116023450_150000_CN_399505633_150000/LConn3 -- bus115/LConn1
  _CN_116023450_150000_CN_109924603_150000/RConn1 -- G_109924603_PLTU_Tello/RConn1 -- _CN_258997962_150000_CN_109924603_150000/LConn1
  _CN_116023450_150000_CN_109924603_150000/RConn2 -- G_109924603_PLTU_Tello/RConn2 -- _CN_258997962_150000_CN_109924603_150000/LConn2
  _CN_116023450_150000_CN_109924603_150000/RConn3 -- G_109924603_PLTU_Tello/RConn3 -- _CN_258997962_150000_CN_109924603_150000/LConn3 -- bus116/LConn1
  T_399505626__/LConn1 -- _CN_116023450_150000_CN_399505626_150000/RConn1
  T_399505626__/LConn2 -- _CN_116023450_150000_CN_399505626_150000/RConn2
  _CN_116023450_150000_CN_399505626_150000/RConn3 -- T_399505626__/LConn3 -- bus117/LConn1
  _CN_116023450_150000_CN_399505633_150000/RConn1 -- T_399505633__/LConn1 -- _CN_399505633_150000_CN_252566435_150000/LConn1
  _CN_116023450_150000_CN_399505633_150000/RConn2 -- T_399505633__/LConn2 -- _CN_399505633_150000_CN_252566435_150000/LConn2
  _CN_116023450_150000_CN_399505633_150000/RConn3 -- T_399505633__/LConn3 -- _CN_399505633_150000_CN_252566435_150000/LConn3 -- bus118/LConn1
  G_399038178_/RConn1 -- _CN_161948315_150000_CN_399038178_150000/RConn1
  G_399038178_/RConn2 -- _CN_161948315_150000_CN_399038178_150000/RConn2
  _CN_161948315_150000_CN_399038178_150000/RConn3 -- G_399038178_/RConn3 -- bus119/LConn1
  T_399038179__/LConn1 -- _CN_161948315_150000_CN_399038179_150000/RConn1
  T_399038179__/LConn2 -- _CN_161948315_150000_CN_399038179_150000/RConn2
  _CN_161948315_150000_CN_399038179_150000/RConn3 -- T_399038179__/LConn3 -- bus120/LConn1
  _CN_311432987_150000_CN_311432989_150000/LConn1 -- T_311432987__Gardu_Induk_Kenjeran/LConn1 -- _CN_311432987_150000_CN_311432990_150000/LConn1
  _CN_311432987_150000_CN_311432989_150000/LConn2 -- T_311432987__Gardu_Induk_Kenjeran/LConn2 -- _CN_311432987_150000_CN_311432990_150000/LConn2
  _CN_311432987_150000_CN_311432989_150000/LConn3 -- T_311432987__Gardu_Induk_Kenjeran/LConn3 -- _CN_311432987_150000_CN_311432990_150000/LConn3 -- bus121/LConn1
  _CN_311432987_150000_CN_311432989_150000/RConn1 -- T_311432989__Gardu_Induk_Sukolilo/LConn1 -- _CN_311432989_150000_CN_311432988_150000/LConn1
  _CN_311432987_150000_CN_311432989_150000/RConn2 -- T_311432989__Gardu_Induk_Sukolilo/LConn2 -- _CN_311432989_150000_CN_311432988_150000/LConn2
  _CN_311432987_150000_CN_311432989_150000/RConn3 -- T_311432989__Gardu_Induk_Sukolilo/LConn3 -- _CN_311432989_150000_CN_311432988_150000/LConn3 -- bus122/LConn1
  T_311432990__Gardu_Induk_Ujung/LConn1 -- _CN_311432987_150000_CN_311432990_150000/RConn1
  T_311432990__Gardu_Induk_Ujung/LConn2 -- _CN_311432987_150000_CN_311432990_150000/RConn2
  _CN_311432987_150000_CN_311432990_150000/RConn3 -- T_311432990__Gardu_Induk_Ujung/LConn3 -- bus123/LConn1
  _CN_311957671_150000_CN_340978681_150000/LConn1 -- T_311957671__Gardu_Induk_Gondang_Wetan/LConn1 -- _CN_311957671_150000_CN_340947951_150000/LConn1
  _CN_311957671_150000_CN_340978681_150000/LConn2 -- T_311957671__Gardu_Induk_Gondang_Wetan/LConn2 -- _CN_311957671_150000_CN_340947951_150000/LConn2
  _CN_311957671_150000_CN_340978681_150000/LConn3 -- T_311957671__Gardu_Induk_Gondang_Wetan/LConn3 -- _CN_311957671_150000_CN_340947951_150000/LConn3 -- bus124/LConn1
  _CN_311957671_150000_CN_340978681_150000/RConn1 -- T_340978681__/RConn1 -- L_340978681/LConn1
  _CN_311957671_150000_CN_340978681_150000/RConn2 -- T_340978681__/RConn2 -- L_340978681/LConn2
  _CN_311957671_150000_CN_340978681_150000/RConn3 -- T_340978681__/RConn3 -- L_340978681/LConn3 -- bus125/LConn1
  _CN_311957671_150000_CN_340947951_150000/RConn1 -- T_340947951__/LConn1 -- _CN_340963798_150000_CN_340947951_150000/RConn1 -- _CN_198149824_150000_CN_340947951_150000/LConn1
  _CN_311957671_150000_CN_340947951_150000/RConn2 -- T_340947951__/LConn2 -- _CN_340963798_150000_CN_340947951_150000/RConn2 -- _CN_198149824_150000_CN_340947951_150000/LConn2
  _CN_311957671_150000_CN_340947951_150000/RConn3 -- T_340947951__/LConn3 -- _CN_340963798_150000_CN_340947951_150000/RConn3 -- bus126/LConn1 -- _CN_198149824_150000_CN_340947951_150000/LConn3
  _CN_399057180_150000_CN_161965853_150000/LConn1 -- T_399057180__/LConn1 -- _CN_399057180_150000_CN_199476032_150000/LConn1 -- _CN_399057180_150000_CN_161969969_150000/LConn1
  _CN_399057180_150000_CN_161965853_150000/LConn2 -- T_399057180__/LConn2 -- _CN_399057180_150000_CN_199476032_150000/LConn2 -- _CN_399057180_150000_CN_161969969_150000/LConn2
  _CN_399057180_150000_CN_161965853_150000/LConn3 -- T_399057180__/LConn3 -- _CN_399057180_150000_CN_199476032_150000/LConn3 -- _CN_399057180_150000_CN_161969969_150000/LConn3 -- bus127/LConn1
  _CN_399057180_150000_CN_161965853_150000/RConn1 -- T_161965853__/RConn1 -- _CN_399057165_150000_CN_161965853_150000/LConn1 -- L_161965853/LConn1
  _CN_399057180_150000_CN_161965853_150000/RConn2 -- T_161965853__/RConn2 -- _CN_399057165_150000_CN_161965853_150000/LConn2 -- L_161965853/LConn2
  _CN_399057180_150000_CN_161965853_150000/RConn3 -- T_161965853__/RConn3 -- _CN_399057165_150000_CN_161965853_150000/LConn3 -- L_161965853/LConn3 -- bus128/LConn1
  T_199476032__/LConn1 -- _CN_399057180_150000_CN_199476032_150000/RConn1
  T_199476032__/LConn2 -- _CN_399057180_150000_CN_199476032_150000/RConn2
  _CN_399057180_150000_CN_199476032_150000/RConn3 -- T_199476032__/LConn3 -- bus129/LConn1
  T_161969969__/LConn1 -- _CN_399057180_150000_CN_161969969_150000/RConn1
  T_161969969__/LConn2 -- _CN_399057180_150000_CN_161969969_150000/RConn2
  _CN_399057180_150000_CN_161969969_150000/RConn3 -- T_161969969__/LConn3 -- bus130/LConn1
  _CN_104412331_150000_CN_265030533_150000/RConn1 -- T_265030533__/LConn1 -- _CN_265030533_150000_CN_265030541_150000/LConn1
  _CN_104412331_150000_CN_265030533_150000/RConn2 -- T_265030533__/LConn2 -- _CN_265030533_150000_CN_265030541_150000/LConn2
  _CN_104412331_150000_CN_265030533_150000/RConn3 -- T_265030533__/LConn3 -- _CN_265030533_150000_CN_265030541_150000/LConn3 -- bus131/LConn1
  T_182845612__/LConn1 -- _CN_182845612_150000_CN_272989134_150000/LConn1
  T_182845612__/LConn2 -- _CN_182845612_150000_CN_272989134_150000/LConn2
  _CN_182845612_150000_CN_272989134_150000/LConn3 -- T_182845612__/LConn3 -- bus132/LConn1
  _CN_182845612_150000_CN_272989134_150000/RConn1 -- T_272989134__/LConn1 -- _CN_269129291_150000_CN_272989134_150000/RConn1
  _CN_182845612_150000_CN_272989134_150000/RConn2 -- T_272989134__/LConn2 -- _CN_269129291_150000_CN_272989134_150000/RConn2
  _CN_182845612_150000_CN_272989134_150000/RConn3 -- T_272989134__/LConn3 -- _CN_269129291_150000_CN_272989134_150000/RConn3 -- bus133/LConn1
  _CN_311432989_150000_CN_311432988_150000/RConn1 -- T_311432988__Gardu_Induk_Rungkut/LConn1 -- _CN_311432988_150000_CN_119360808_150000/LConn1 -- _CN_166644946_150000_CN_311432988_150000/RConn1
  _CN_311432989_150000_CN_311432988_150000/RConn2 -- T_311432988__Gardu_Induk_Rungkut/LConn2 -- _CN_311432988_150000_CN_119360808_150000/LConn2 -- _CN_166644946_150000_CN_311432988_150000/RConn2
  _CN_311432989_150000_CN_311432988_150000/RConn3 -- T_311432988__Gardu_Induk_Rungkut/LConn3 -- _CN_311432988_150000_CN_119360808_150000/LConn3 -- bus134/LConn1 -- _CN_166644946_150000_CN_311432988_150000/RConn3
  _CN_189064370_150000_CN_398892599_150000/LConn1 -- T_189064370__Gardu_Induk_Situbondo_(PLN)/LConn1 -- _CN_189064370_150000_CN_299352934_150000/LConn1 -- _CN_189064370_150000_CN_186337693_150000/LConn1 -- _CN_189064370_150000_CN_339796951_150000/LConn1
  _CN_189064370_150000_CN_398892599_150000/LConn2 -- T_189064370__Gardu_Induk_Situbondo_(PLN)/LConn2 -- _CN_189064370_150000_CN_299352934_150000/LConn2 -- _CN_189064370_150000_CN_186337693_150000/LConn2 -- _CN_189064370_150000_CN_339796951_150000/LConn2
  _CN_189064370_150000_CN_398892599_150000/LConn3 -- T_189064370__Gardu_Induk_Situbondo_(PLN)/LConn3 -- _CN_189064370_150000_CN_299352934_150000/LConn3 -- bus135/LConn1 -- _CN_189064370_150000_CN_186337693_150000/LConn3 -- _CN_189064370_150000_CN_339796951_150000/LConn3
  _CN_189064370_150000_CN_398892599_150000/RConn1 -- T_398892599__/LConn1 -- _CN_157804728_150000_CN_398892599_150000/LConn1
  _CN_189064370_150000_CN_398892599_150000/RConn2 -- T_398892599__/LConn2 -- _CN_157804728_150000_CN_398892599_150000/LConn2
  _CN_189064370_150000_CN_398892599_150000/RConn3 -- T_398892599__/LConn3 -- _CN_157804728_150000_CN_398892599_150000/LConn3 -- bus136/LConn1
  _CN_189064370_150000_CN_186337693_150000/RConn1 -- T_186337693__Gardu_Induk_Banyuwangi/LConn1 -- _CN_157804728_150000_CN_186337693_150000/LConn1 -- _CN_339796951_150000_CN_186337693_150000/LConn1
  _CN_189064370_150000_CN_186337693_150000/RConn2 -- T_186337693__Gardu_Induk_Banyuwangi/LConn2 -- _CN_157804728_150000_CN_186337693_150000/LConn2 -- _CN_339796951_150000_CN_186337693_150000/LConn2
  _CN_189064370_150000_CN_186337693_150000/RConn3 -- T_186337693__Gardu_Induk_Banyuwangi/LConn3 -- _CN_157804728_150000_CN_186337693_150000/LConn3 -- _CN_339796951_150000_CN_186337693_150000/LConn3 -- bus137/LConn1
  _CN_189064370_150000_CN_339796951_150000/RConn1 -- T_339796951__/LConn1 -- _CN_339796951_150000_CN_186337693_150000/RConn1
  _CN_189064370_150000_CN_339796951_150000/RConn2 -- T_339796951__/LConn2 -- _CN_339796951_150000_CN_186337693_150000/RConn2
  _CN_189064370_150000_CN_339796951_150000/RConn3 -- T_339796951__/LConn3 -- _CN_339796951_150000_CN_186337693_150000/RConn3 -- bus138/LConn1
  _CN_189064370_150000_CN_299352934_150000/RConn1 -- T_299352934__/RConn1 -- _CN_299352934_150000_CN_340963798_150000/RConn1 -- L_299352934/LConn1
  _CN_189064370_150000_CN_299352934_150000/RConn2 -- T_299352934__/RConn2 -- _CN_299352934_150000_CN_340963798_150000/RConn2 -- L_299352934/LConn2
  _CN_189064370_150000_CN_299352934_150000/RConn3 -- T_299352934__/RConn3 -- _CN_299352934_150000_CN_340963798_150000/RConn3 -- L_299352934/LConn3 -- bus139/LConn1
  _CN_268831411_150000_CN_268865913_150000/RConn1 -- T_268865913__/LConn1 -- _CN_268865913_150000_CN_268865917_150000/RConn1
  _CN_268831411_150000_CN_268865913_150000/RConn2 -- T_268865913__/LConn2 -- _CN_268865913_150000_CN_268865917_150000/RConn2
  _CN_268831411_150000_CN_268865913_150000/RConn3 -- T_268865913__/LConn3 -- _CN_268865913_150000_CN_268865917_150000/RConn3 -- bus140/LConn1
  _CN_399714486_150000_CN_257725651_150000/LConn1 -- T_399714486__/LConn1 -- _CN_399714486_150000_CN_244815736_150000/LConn1
  _CN_399714486_150000_CN_257725651_150000/LConn2 -- T_399714486__/LConn2 -- _CN_399714486_150000_CN_244815736_150000/LConn2
  _CN_399714486_150000_CN_257725651_150000/LConn3 -- T_399714486__/LConn3 -- _CN_399714486_150000_CN_244815736_150000/LConn3 -- bus141/LConn1
  T_257725651__/LConn1 -- _CN_399714486_150000_CN_257725651_150000/RConn1
  T_257725651__/LConn2 -- _CN_399714486_150000_CN_257725651_150000/RConn2
  _CN_399714486_150000_CN_257725651_150000/RConn3 -- T_257725651__/LConn3 -- bus142/LConn1
  T_244815736__/LConn1 -- _CN_399714486_150000_CN_244815736_150000/RConn1
  T_244815736__/LConn2 -- _CN_399714486_150000_CN_244815736_150000/RConn2
  _CN_399714486_150000_CN_244815736_150000/RConn3 -- T_244815736__/LConn3 -- bus143/LConn1
  _CN_157804728_150000_CN_186337693_150000/RConn1 -- T_157804728__/LConn1 -- _CN_157804728_150000_CN_398892599_150000/RConn1 -- _CN_157804728_150000_CN_198149824_150000/LConn1
  _CN_157804728_150000_CN_186337693_150000/RConn2 -- T_157804728__/LConn2 -- _CN_157804728_150000_CN_398892599_150000/RConn2 -- _CN_157804728_150000_CN_198149824_150000/LConn2
  _CN_157804728_150000_CN_186337693_150000/RConn3 -- T_157804728__/LConn3 -- _CN_157804728_150000_CN_398892599_150000/RConn3 -- bus144/LConn1 -- _CN_157804728_150000_CN_198149824_150000/LConn3
  _CN_157804728_150000_CN_198149824_150000/RConn1 -- T_198149824_500000_Gardu_Listrik/LConn1 -- _CN_198149824_150000_CN_340947951_150000/RConn1
  _CN_157804728_150000_CN_198149824_150000/RConn2 -- T_198149824_500000_Gardu_Listrik/LConn2 -- _CN_198149824_150000_CN_340947951_150000/RConn2
  _CN_157804728_150000_CN_198149824_150000/RConn3 -- T_198149824_500000_Gardu_Listrik/LConn3 -- _CN_198149824_150000_CN_340947951_150000/RConn3 -- bus145/LConn1
  T_249207412__/LConn1 -- _CN_249207412_150000_CN_277204262_150000/LConn1
  T_249207412__/LConn2 -- _CN_249207412_150000_CN_277204262_150000/LConn2
  _CN_249207412_150000_CN_277204262_150000/LConn3 -- T_249207412__/LConn3 -- bus146/LConn1
  _CN_249207412_150000_CN_277204262_150000/RConn1 -- T_277204262__/LConn1 -- _CN_277204263_150000_CN_277204262_150000/RConn1 -- _CN_277183761_150000_CN_277204262_150000/LConn1
  _CN_249207412_150000_CN_277204262_150000/RConn2 -- T_277204262__/LConn2 -- _CN_277204263_150000_CN_277204262_150000/RConn2 -- _CN_277183761_150000_CN_277204262_150000/LConn2
  _CN_249207412_150000_CN_277204262_150000/RConn3 -- T_277204262__/LConn3 -- _CN_277204263_150000_CN_277204262_150000/RConn3 -- _CN_277183761_150000_CN_277204262_150000/LConn3 -- bus147/LConn1
  T_261184996__/LConn1 -- _CN_269160480_150000_CN_261184996_150000/RConn1
  T_261184996__/LConn2 -- _CN_269160480_150000_CN_261184996_150000/RConn2
  _CN_269160480_150000_CN_261184996_150000/RConn3 -- T_261184996__/LConn3 -- bus148/LConn1
  T_398909635__/LConn1 -- _CN_398909635_150000_CN_352100214_150000/LConn1
  T_398909635__/LConn2 -- _CN_398909635_150000_CN_352100214_150000/LConn2
  _CN_398909635_150000_CN_352100214_150000/LConn3 -- T_398909635__/LConn3 -- bus149/LConn1
  _CN_398909635_150000_CN_352100214_150000/RConn1 -- T_352100214__/LConn1 -- _CN_398972213_150000_CN_352100214_150000/LConn1
  _CN_398909635_150000_CN_352100214_150000/RConn2 -- T_352100214__/LConn2 -- _CN_398972213_150000_CN_352100214_150000/LConn2
  _CN_398909635_150000_CN_352100214_150000/RConn3 -- T_352100214__/LConn3 -- _CN_398972213_150000_CN_352100214_150000/LConn3 -- bus150/LConn1
  T_166699717__/LConn1 -- _CN_166699717_150000_CN_265923575_150000/RConn1
  T_166699717__/LConn2 -- _CN_166699717_150000_CN_265923575_150000/RConn2
  _CN_166699717_150000_CN_265923575_150000/RConn3 -- T_166699717__/LConn3 -- bus151/LConn1
  T_339792673__/LConn1 -- _CN_339792673_150000_CN_339792684_150000/RConn1
  T_339792673__/LConn2 -- _CN_339792673_150000_CN_339792684_150000/RConn2
  _CN_339792673_150000_CN_339792684_150000/RConn3 -- T_339792673__/LConn3 -- bus152/LConn1
  T_258997962__Gardu_Induk_PLN/LConn1 -- _CN_258997962_150000_CN_109924603_150000/RConn1
  T_258997962__Gardu_Induk_PLN/LConn2 -- _CN_258997962_150000_CN_109924603_150000/RConn2
  _CN_258997962_150000_CN_109924603_150000/RConn3 -- T_258997962__Gardu_Induk_PLN/LConn3 -- bus153/LConn1
  _CN_166644946_150000_CN_340978671_150000/RConn1 -- T_340978671__/LConn1 -- _CN_398972213_150000_CN_340978671_150000/LConn1 -- _CN_340978671_150000_CN_340978685_150000/LConn1
  _CN_166644946_150000_CN_340978671_150000/RConn2 -- T_340978671__/LConn2 -- _CN_398972213_150000_CN_340978671_150000/LConn2 -- _CN_340978671_150000_CN_340978685_150000/LConn2
  _CN_166644946_150000_CN_340978671_150000/RConn3 -- T_340978671__/LConn3 -- _CN_398972213_150000_CN_340978671_150000/LConn3 -- _CN_340978671_150000_CN_340978685_150000/LConn3 -- bus154/LConn1
  T_311963425__Gardu_Induk_Darmo_Grande/LConn1 -- _CN_166644946_150000_CN_311963425_150000/RConn1
  T_311963425__Gardu_Induk_Darmo_Grande/LConn2 -- _CN_166644946_150000_CN_311963425_150000/RConn2
  _CN_166644946_150000_CN_311963425_150000/RConn3 -- T_311963425__Gardu_Induk_Darmo_Grande/LConn3 -- bus155/LConn1
  T_311963427__Gardu_Induk_Karang_Pilang/LConn1 -- _CN_166644946_150000_CN_311963427_150000/RConn1
  T_311963427__Gardu_Induk_Karang_Pilang/LConn2 -- _CN_166644946_150000_CN_311963427_150000/RConn2
  _CN_166644946_150000_CN_311963427_150000/RConn3 -- T_311963427__Gardu_Induk_Karang_Pilang/LConn3 -- bus156/LConn1
  T_398787876__/LConn1 -- _CN_398787876_150000_CN_309311292_150000/LConn1
  T_398787876__/LConn2 -- _CN_398787876_150000_CN_309311292_150000/LConn2
  _CN_398787876_150000_CN_309311292_150000/LConn3 -- T_398787876__/LConn3 -- bus157/LConn1
  T_309311292__Gardu_Induk_Lamreung/LConn1 -- _CN_398787876_150000_CN_309311292_150000/RConn1
  T_309311292__Gardu_Induk_Lamreung/LConn2 -- _CN_398787876_150000_CN_309311292_150000/RConn2
  _CN_398787876_150000_CN_309311292_150000/RConn3 -- T_309311292__Gardu_Induk_Lamreung/LConn3 -- bus158/LConn1
  T_161963229__/LConn1 -- _CN_161963229_150000_CN_161960924_150000/LConn1
  T_161963229__/LConn2 -- _CN_161963229_150000_CN_161960924_150000/LConn2
  _CN_161963229_150000_CN_161960924_150000/LConn3 -- T_161963229__/LConn3 -- bus159/LConn1
  _CN_161963229_150000_CN_161960924_150000/RConn1 -- T_161960924__/RConn1 -- L_161960924/LConn1
  _CN_161963229_150000_CN_161960924_150000/RConn2 -- T_161960924__/RConn2 -- L_161960924/LConn2
  _CN_161963229_150000_CN_161960924_150000/RConn3 -- T_161960924__/RConn3 -- L_161960924/LConn3 -- bus160/LConn1
  T_252566435__GARDU_INDUK_PLN/LConn1 -- _CN_399505633_150000_CN_252566435_150000/RConn1
  T_252566435__GARDU_INDUK_PLN/LConn2 -- _CN_399505633_150000_CN_252566435_150000/RConn2
  _CN_399505633_150000_CN_252566435_150000/RConn3 -- T_252566435__GARDU_INDUK_PLN/LConn3 -- bus161/LConn1
  _CN_277204263_150000_CN_277183760_150000/RConn1 -- T_277183760__/LConn1 -- _CN_277183760_150000_CN_277204260_150000/LConn1
  _CN_277204263_150000_CN_277183760_150000/RConn2 -- T_277183760__/LConn2 -- _CN_277183760_150000_CN_277204260_150000/LConn2
  _CN_277204263_150000_CN_277183760_150000/RConn3 -- T_277183760__/LConn3 -- _CN_277183760_150000_CN_277204260_150000/LConn3 -- bus162/LConn1
  _CN_265002738_150000_CN_265002740_150000/LConn1 -- T_265002738__/LConn1 -- _CN_265002738_150000_CN_279284589_150000/RConn1
  _CN_265002738_150000_CN_265002740_150000/LConn2 -- T_265002738__/LConn2 -- _CN_265002738_150000_CN_279284589_150000/RConn2
  _CN_265002738_150000_CN_265002740_150000/LConn3 -- T_265002738__/LConn3 -- _CN_265002738_150000_CN_279284589_150000/RConn3 -- bus163/LConn1
  T_265002740__/LConn1 -- _CN_265002738_150000_CN_265002740_150000/RConn1
  T_265002740__/LConn2 -- _CN_265002738_150000_CN_265002740_150000/RConn2
  _CN_265002738_150000_CN_265002740_150000/RConn3 -- T_265002740__/LConn3 -- bus164/LConn1
  _CN_311666430_150000_CN_311666433_150000/RConn1 -- T_311666433__Gardu_Induk_Sampang/LConn1 -- _CN_311666432_150000_CN_311666433_150000/LConn1
  _CN_311666430_150000_CN_311666433_150000/RConn2 -- T_311666433__Gardu_Induk_Sampang/LConn2 -- _CN_311666432_150000_CN_311666433_150000/LConn2
  _CN_311666430_150000_CN_311666433_150000/RConn3 -- T_311666433__Gardu_Induk_Sampang/LConn3 -- _CN_311666432_150000_CN_311666433_150000/LConn3 -- bus165/LConn1
  _CN_311666432_150000_CN_311666434_150000/LConn1 -- T_311666432__Gardu_Induk_Pamekasan/LConn1 -- _CN_311666432_150000_CN_311666433_150000/RConn1
  _CN_311666432_150000_CN_311666434_150000/LConn2 -- T_311666432__Gardu_Induk_Pamekasan/LConn2 -- _CN_311666432_150000_CN_311666433_150000/RConn2
  _CN_311666432_150000_CN_311666434_150000/LConn3 -- T_311666432__Gardu_Induk_Pamekasan/LConn3 -- _CN_311666432_150000_CN_311666433_150000/RConn3 -- bus166/LConn1
  T_311666434__Gardu_Induk_Sumenep/LConn1 -- _CN_311666432_150000_CN_311666434_150000/RConn1
  T_311666434__Gardu_Induk_Sumenep/LConn2 -- _CN_311666432_150000_CN_311666434_150000/RConn2
  _CN_311666432_150000_CN_311666434_150000/RConn3 -- T_311666434__Gardu_Induk_Sumenep/LConn3 -- bus167/LConn1
  G_269508907_Cibatu/RConn1 -- _CN_271376043_150000_CN_269508907_150000/RConn1
  G_269508907_Cibatu/RConn2 -- _CN_271376043_150000_CN_269508907_150000/RConn2
  _CN_271376043_150000_CN_269508907_150000/RConn3 -- G_269508907_Cibatu/RConn3 -- bus168/LConn1
  _CN_271376043_150000_CN_153303534_150000/RConn1 -- T_153303534__PLT/LConn1 -- _CN_264713279_150000_CN_153303534_150000/RConn1
  _CN_271376043_150000_CN_153303534_150000/RConn2 -- T_153303534__PLT/LConn2 -- _CN_264713279_150000_CN_153303534_150000/RConn2
  _CN_271376043_150000_CN_153303534_150000/RConn3 -- T_153303534__PLT/LConn3 -- _CN_264713279_150000_CN_153303534_150000/RConn3 -- bus169/LConn1
  _CN_399057165_150000_CN_264106354_150000/LConn1 -- T_399057165__/LConn1 -- _CN_399057165_150000_CN_161965853_150000/RConn1 -- _CN_399057165_150000_CN_399057172_150000/RConn1
  _CN_399057165_150000_CN_264106354_150000/LConn2 -- T_399057165__/LConn2 -- _CN_399057165_150000_CN_161965853_150000/RConn2 -- _CN_399057165_150000_CN_399057172_150000/RConn2
  _CN_399057165_150000_CN_264106354_150000/LConn3 -- T_399057165__/LConn3 -- _CN_399057165_150000_CN_161965853_150000/RConn3 -- _CN_399057165_150000_CN_399057172_150000/RConn3 -- bus170/LConn1
  T_264106354__/LConn1 -- _CN_399057165_150000_CN_264106354_150000/RConn1
  T_264106354__/LConn2 -- _CN_399057165_150000_CN_264106354_150000/RConn2
  _CN_399057165_150000_CN_264106354_150000/RConn3 -- T_264106354__/LConn3 -- bus171/LConn1
  T_277204260__/LConn1 -- _CN_277183760_150000_CN_277204260_150000/RConn1
  T_277204260__/LConn2 -- _CN_277183760_150000_CN_277204260_150000/RConn2
  _CN_277183760_150000_CN_277204260_150000/RConn3 -- T_277204260__/LConn3 -- bus172/LConn1
  _CN_277183761_150000_CN_277204262_150000/RConn1 -- T_277183761__/LConn1 -- _CN_277183761_150000_CN_340205049_150000/RConn1
  _CN_277183761_150000_CN_277204262_150000/RConn2 -- T_277183761__/LConn2 -- _CN_277183761_150000_CN_340205049_150000/RConn2
  _CN_277183761_150000_CN_277204262_150000/RConn3 -- T_277183761__/LConn3 -- _CN_277183761_150000_CN_340205049_150000/RConn3 -- bus173/LConn1
  T_271678852__/LConn1 -- _CN_269468436_150000_CN_271678852_150000/RConn1
  T_271678852__/LConn2 -- _CN_269468436_150000_CN_271678852_150000/RConn2
  _CN_269468436_150000_CN_271678852_150000/RConn3 -- T_271678852__/LConn3 -- bus174/LConn1
  T_119360808__Gardu_Induk_Wonorejo/LConn1 -- _CN_311432988_150000_CN_119360808_150000/RConn1
  T_119360808__Gardu_Induk_Wonorejo/LConn2 -- _CN_311432988_150000_CN_119360808_150000/RConn2
  _CN_311432988_150000_CN_119360808_150000/RConn3 -- T_119360808__Gardu_Induk_Wonorejo/LConn3 -- bus175/LConn1
  T_339792680__/LConn1 -- _CN_339792684_150000_CN_339792680_150000/RConn1
  T_339792680__/LConn2 -- _CN_339792684_150000_CN_339792680_150000/RConn2
  _CN_339792684_150000_CN_339792680_150000/RConn3 -- T_339792680__/LConn3 -- bus176/LConn1
  T_185683916__/LConn1 -- _CN_339792684_150000_CN_185683916_150000/RConn1
  T_185683916__/LConn2 -- _CN_339792684_150000_CN_185683916_150000/RConn2
  _CN_339792684_150000_CN_185683916_150000/RConn3 -- T_185683916__/LConn3 -- bus177/LConn1
  T_339792685__/LConn1 -- _CN_339792684_150000_CN_339792685_150000/RConn1
  T_339792685__/LConn2 -- _CN_339792684_150000_CN_339792685_150000/RConn2
  _CN_339792684_150000_CN_339792685_150000/RConn3 -- T_339792685__/LConn3 -- bus178/LConn1
  _CN_398972213_150000_CN_352100214_150000/RConn1 -- T_398972213__/LConn1 -- _CN_398972213_150000_CN_340978671_150000/RConn1
  _CN_398972213_150000_CN_352100214_150000/RConn2 -- T_398972213__/LConn2 -- _CN_398972213_150000_CN_340978671_150000/RConn2
  _CN_398972213_150000_CN_352100214_150000/RConn3 -- T_398972213__/LConn3 -- _CN_398972213_150000_CN_340978671_150000/RConn3 -- bus179/LConn1
  _CN_265030532_150000_CN_270788980_150000/LConn1 -- T_265030532__/LConn1 -- _CN_265030532_150000_CN_265030541_150000/LConn1
  _CN_265030532_150000_CN_270788980_150000/LConn2 -- T_265030532__/LConn2 -- _CN_265030532_150000_CN_265030541_150000/LConn2
  _CN_265030532_150000_CN_270788980_150000/LConn3 -- T_265030532__/LConn3 -- _CN_265030532_150000_CN_265030541_150000/LConn3 -- bus180/LConn1
  G_270788980_/RConn1 -- _CN_265030532_150000_CN_270788980_150000/RConn1
  G_270788980_/RConn2 -- _CN_265030532_150000_CN_270788980_150000/RConn2
  _CN_265030532_150000_CN_270788980_150000/RConn3 -- G_270788980_/RConn3 -- bus181/LConn1
  _CN_265030532_150000_CN_265030541_150000/RConn1 -- T_265030541__/LConn1 -- _CN_265030533_150000_CN_265030541_150000/RConn1
  _CN_265030532_150000_CN_265030541_150000/RConn2 -- T_265030541__/LConn2 -- _CN_265030533_150000_CN_265030541_150000/RConn2
  _CN_265030532_150000_CN_265030541_150000/RConn3 -- T_265030541__/LConn3 -- _CN_265030533_150000_CN_265030541_150000/RConn3 -- bus182/LConn1
  T_340978685__/LConn1 -- _CN_340978671_150000_CN_340978685_150000/RConn1
  T_340978685__/LConn2 -- _CN_340978671_150000_CN_340978685_150000/RConn2
  _CN_340978671_150000_CN_340978685_150000/RConn3 -- T_340978685__/LConn3 -- bus183/LConn1
  T_271991718__Gardu_Induk_Indonesia_Power/LConn1 -- _CN_271991718_150000_CN_253654957_150000/LConn1
  T_271991718__Gardu_Induk_Indonesia_Power/LConn2 -- _CN_271991718_150000_CN_253654957_150000/LConn2
  _CN_271991718_150000_CN_253654957_150000/LConn3 -- T_271991718__Gardu_Induk_Indonesia_Power/LConn3 -- bus184/LConn1
  T_253654957__/LConn1 -- _CN_271991718_150000_CN_253654957_150000/RConn1
  T_253654957__/LConn2 -- _CN_271991718_150000_CN_253654957_150000/RConn2
  _CN_271991718_150000_CN_253654957_150000/RConn3 -- T_253654957__/LConn3 -- bus185/LConn1
  T_261185003__/LConn1 -- _CN_264719089_150000_CN_261185003_150000/RConn1
  T_261185003__/LConn2 -- _CN_264719089_150000_CN_261185003_150000/RConn2
  _CN_264719089_150000_CN_261185003_150000/RConn3 -- T_261185003__/LConn3 -- bus186/LConn1
  T_399094735__/LConn1 -- _CN_269129291_150000_CN_399094735_150000/RConn1
  T_399094735__/LConn2 -- _CN_269129291_150000_CN_399094735_150000/RConn2
  _CN_269129291_150000_CN_399094735_150000/RConn3 -- T_399094735__/LConn3 -- bus187/LConn1
  T_269490135__/LConn1 -- _CN_269490135_150000_CN_269490147_150000/RConn1
  T_269490135__/LConn2 -- _CN_269490135_150000_CN_269490147_150000/RConn2
  _CN_269490135_150000_CN_269490147_150000/RConn3 -- T_269490135__/LConn3 -- bus188/LConn1
  _CN_265568001_500000_CN_340978681_500000/LConn1 -- T_265568001__GITET_Krian/LConn1 -- _CN_265568001_500000_CN_398909640_500000/LConn1 -- _CN_265568001_500000_CN_166633831_500000/LConn1 -- _CN_265568001_500000_CN_311479837_500000/LConn1
  _CN_265568001_500000_CN_340978681_500000/LConn2 -- T_265568001__GITET_Krian/LConn2 -- _CN_265568001_500000_CN_398909640_500000/LConn2 -- _CN_265568001_500000_CN_166633831_500000/LConn2 -- _CN_265568001_500000_CN_311479837_500000/LConn2
  _CN_265568001_500000_CN_340978681_500000/LConn3 -- T_265568001__GITET_Krian/LConn3 -- _CN_265568001_500000_CN_398909640_500000/LConn3 -- _CN_265568001_500000_CN_166633831_500000/LConn3 -- _CN_265568001_500000_CN_311479837_500000/LConn3 -- bus189/LConn1
  _CN_265568001_500000_CN_340978681_500000/RConn1 -- T_340978681__/LConn1 -- _CN_265318414_500000_CN_340978681_500000/LConn1
  _CN_265568001_500000_CN_340978681_500000/RConn2 -- T_340978681__/LConn2 -- _CN_265318414_500000_CN_340978681_500000/LConn2
  _CN_265568001_500000_CN_340978681_500000/RConn3 -- T_340978681__/LConn3 -- _CN_265318414_500000_CN_340978681_500000/LConn3 -- bus190/LConn1
  T_398909640__/LConn1 -- _CN_265568001_500000_CN_398909640_500000/RConn1
  T_398909640__/LConn2 -- _CN_265568001_500000_CN_398909640_500000/RConn2
  _CN_265568001_500000_CN_398909640_500000/RConn3 -- T_398909640__/LConn3 -- bus191/LConn1
  _CN_265568001_500000_CN_166633831_500000/RConn1 -- T_166633831__/LConn1 -- _CN_166633831_500000_CN_195105317_500000/LConn1 -- _CN_166633831_500000_CN_261185002_500000/LConn1 -- _CN_104339545_500000_CN_166633831_500000/LConn1
  _CN_265568001_500000_CN_166633831_500000/RConn2 -- T_166633831__/LConn2 -- _CN_166633831_500000_CN_195105317_500000/LConn2 -- _CN_166633831_500000_CN_261185002_500000/LConn2 -- _CN_104339545_500000_CN_166633831_500000/LConn2
  _CN_265568001_500000_CN_166633831_500000/RConn3 -- T_166633831__/LConn3 -- _CN_166633831_500000_CN_195105317_500000/LConn3 -- bus192/LConn1 -- _CN_166633831_500000_CN_261185002_500000/LConn3 -- _CN_104339545_500000_CN_166633831_500000/LConn3
  T_311479837__GITET_Gresik/LConn1 -- _CN_265568001_500000_CN_311479837_500000/RConn1
  T_311479837__GITET_Gresik/LConn2 -- _CN_265568001_500000_CN_311479837_500000/RConn2
  _CN_265568001_500000_CN_311479837_500000/RConn3 -- T_311479837__GITET_Gresik/LConn3 -- bus193/LConn1
  T_399100034__/LConn1 -- _CN_399100034_500000_CN_399100035_500000/LConn1
  T_399100034__/LConn2 -- _CN_399100034_500000_CN_399100035_500000/LConn2
  _CN_399100034_500000_CN_399100035_500000/LConn3 -- T_399100034__/LConn3 -- bus194/LConn1
  _CN_399100034_500000_CN_399100035_500000/RConn1 -- T_399100035__/LConn1 -- _CN_399100035_500000_CN_264550744_500000/LConn1
  _CN_399100034_500000_CN_399100035_500000/RConn2 -- T_399100035__/LConn2 -- _CN_399100035_500000_CN_264550744_500000/LConn2
  _CN_399100034_500000_CN_399100035_500000/RConn3 -- T_399100035__/LConn3 -- _CN_399100035_500000_CN_264550744_500000/LConn3 -- bus195/LConn1
  T_399022979__/LConn1 -- _CN_399022979_500000_CN_271376037_500000/LConn1
  T_399022979__/LConn2 -- _CN_399022979_500000_CN_271376037_500000/LConn2
  _CN_399022979_500000_CN_271376037_500000/LConn3 -- T_399022979__/LConn3 -- bus196/LConn1
  T_271376037__/LConn1 -- _CN_399022979_500000_CN_271376037_500000/RConn1
  T_271376037__/LConn2 -- _CN_399022979_500000_CN_271376037_500000/RConn2
  _CN_399022979_500000_CN_271376037_500000/RConn3 -- T_271376037__/LConn3 -- bus197/LConn1
  _CN_265318414_500000_CN_299352934_500000/LConn1 -- T_265318414__/LConn1 -- _CN_265318414_500000_CN_104339545_500000/LConn1 -- _CN_265318414_500000_CN_340978681_500000/RConn1
  _CN_265318414_500000_CN_299352934_500000/LConn2 -- T_265318414__/LConn2 -- _CN_265318414_500000_CN_104339545_500000/LConn2 -- _CN_265318414_500000_CN_340978681_500000/RConn2
  _CN_265318414_500000_CN_299352934_500000/LConn3 -- T_265318414__/LConn3 -- _CN_265318414_500000_CN_104339545_500000/LConn3 -- bus198/LConn1 -- _CN_265318414_500000_CN_340978681_500000/RConn3
  _CN_265318414_500000_CN_299352934_500000/RConn1 -- T_299352934__/LConn1 -- _CN_299352934_500000_CN_340912781_500000/LConn1
  _CN_265318414_500000_CN_299352934_500000/RConn2 -- T_299352934__/LConn2 -- _CN_299352934_500000_CN_340912781_500000/LConn2
  _CN_265318414_500000_CN_299352934_500000/RConn3 -- T_299352934__/LConn3 -- _CN_299352934_500000_CN_340912781_500000/LConn3 -- bus199/LConn1
  _CN_265318414_500000_CN_104339545_500000/RConn1 -- T_104339545__/LConn1 -- _CN_267626657_500000_CN_104339545_500000/LConn1 -- _CN_104339545_500000_CN_166633831_500000/RConn1
  _CN_265318414_500000_CN_104339545_500000/RConn2 -- T_104339545__/LConn2 -- _CN_267626657_500000_CN_104339545_500000/LConn2 -- _CN_104339545_500000_CN_166633831_500000/RConn2
  _CN_265318414_500000_CN_104339545_500000/RConn3 -- T_104339545__/LConn3 -- _CN_267626657_500000_CN_104339545_500000/LConn3 -- _CN_104339545_500000_CN_166633831_500000/RConn3 -- bus200/LConn1
  _CN_399100035_500000_CN_264550744_500000/RConn1 -- T_264550744__/LConn1 -- _CN_264713291_500000_CN_264550744_500000/LConn1 -- _CN_264550744_500000_CN_264410236_500000/LConn1
  _CN_399100035_500000_CN_264550744_500000/RConn2 -- T_264550744__/LConn2 -- _CN_264713291_500000_CN_264550744_500000/LConn2 -- _CN_264550744_500000_CN_264410236_500000/LConn2
  _CN_399100035_500000_CN_264550744_500000/RConn3 -- T_264550744__/LConn3 -- _CN_264713291_500000_CN_264550744_500000/LConn3 -- _CN_264550744_500000_CN_264410236_500000/LConn3 -- bus201/LConn1
  T_267626657__/LConn1 -- _CN_267626657_500000_CN_104339545_500000/RConn1
  T_267626657__/LConn2 -- _CN_267626657_500000_CN_104339545_500000/RConn2
  _CN_267626657_500000_CN_104339545_500000/RConn3 -- T_267626657__/LConn3 -- bus202/LConn1
  T_161965853__/LConn1 -- _CN_161965853_500000_CN_199476040_500000/LConn1
  T_161965853__/LConn2 -- _CN_161965853_500000_CN_199476040_500000/LConn2
  _CN_161965853_500000_CN_199476040_500000/LConn3 -- T_161965853__/LConn3 -- bus203/LConn1
  _CN_161965853_500000_CN_199476040_500000/RConn1 -- T_199476040__/LConn1 -- _CN_199476040_500000_CN_169444592_500000/LConn1
  _CN_161965853_500000_CN_199476040_500000/RConn2 -- T_199476040__/LConn2 -- _CN_199476040_500000_CN_169444592_500000/LConn2
  _CN_161965853_500000_CN_199476040_500000/RConn3 -- T_199476040__/LConn3 -- _CN_199476040_500000_CN_169444592_500000/LConn3 -- bus204/LConn1
  _CN_199476040_500000_CN_169444592_500000/RConn1 -- T_169444592__/LConn1 -- _CN_161960933_500000_CN_169444592_500000/LConn1
  _CN_199476040_500000_CN_169444592_500000/RConn2 -- T_169444592__/LConn2 -- _CN_161960933_500000_CN_169444592_500000/LConn2
  _CN_199476040_500000_CN_169444592_500000/RConn3 -- T_169444592__/LConn3 -- _CN_161960933_500000_CN_169444592_500000/LConn3 -- bus205/LConn1
  _CN_264713291_500000_CN_161960924_500000/LConn1 -- T_264713291__/LConn1 -- _CN_264713291_500000_CN_264550744_500000/RConn1
  _CN_264713291_500000_CN_161960924_500000/LConn2 -- T_264713291__/LConn2 -- _CN_264713291_500000_CN_264550744_500000/RConn2
  _CN_264713291_500000_CN_161960924_500000/LConn3 -- T_264713291__/LConn3 -- _CN_264713291_500000_CN_264550744_500000/RConn3 -- bus206/LConn1
  _CN_264713291_500000_CN_161960924_500000/RConn1 -- T_161960924__/LConn1 -- _CN_161960924_500000_CN_161960933_500000/LConn1
  _CN_264713291_500000_CN_161960924_500000/RConn2 -- T_161960924__/LConn2 -- _CN_161960924_500000_CN_161960933_500000/LConn2
  _CN_264713291_500000_CN_161960924_500000/RConn3 -- T_161960924__/LConn3 -- _CN_161960924_500000_CN_161960933_500000/LConn3 -- bus207/LConn1
  _CN_264550744_500000_CN_264410236_500000/RConn1 -- T_264410236__/LConn1 -- _CN_261185002_500000_CN_264410236_500000/LConn1
  _CN_264550744_500000_CN_264410236_500000/RConn2 -- T_264410236__/LConn2 -- _CN_261185002_500000_CN_264410236_500000/LConn2
  _CN_264550744_500000_CN_264410236_500000/RConn3 -- T_264410236__/LConn3 -- _CN_261185002_500000_CN_264410236_500000/LConn3 -- bus208/LConn1
  _CN_161960924_500000_CN_161960933_500000/RConn1 -- T_161960933__/LConn1 -- _CN_399038181_500000_CN_161960933_500000/LConn1 -- _CN_161960933_500000_CN_169444592_500000/RConn1
  _CN_161960924_500000_CN_161960933_500000/RConn2 -- T_161960933__/LConn2 -- _CN_399038181_500000_CN_161960933_500000/LConn2 -- _CN_161960933_500000_CN_169444592_500000/RConn2
  _CN_161960924_500000_CN_161960933_500000/RConn3 -- T_161960933__/LConn3 -- _CN_399038181_500000_CN_161960933_500000/LConn3 -- _CN_161960933_500000_CN_169444592_500000/RConn3 -- bus209/LConn1
  T_399038181__/LConn1 -- _CN_399038181_500000_CN_161960933_500000/RConn1
  T_399038181__/LConn2 -- _CN_399038181_500000_CN_161960933_500000/RConn2
  _CN_399038181_500000_CN_161960933_500000/RConn3 -- T_399038181__/LConn3 -- bus210/LConn1
  G_340912781_/RConn1 -- _CN_299352934_500000_CN_340912781_500000/RConn1
  G_340912781_/RConn2 -- _CN_299352934_500000_CN_340912781_500000/RConn2
  _CN_299352934_500000_CN_340912781_500000/RConn3 -- G_340912781_/RConn3 -- bus211/LConn1
  _CN_166633831_500000_CN_261185002_500000/RConn1 -- T_261185002__/LConn1 -- _CN_261185002_500000_CN_264410236_500000/RConn1
  _CN_166633831_500000_CN_261185002_500000/RConn2 -- T_261185002__/LConn2 -- _CN_261185002_500000_CN_264410236_500000/RConn2
  _CN_166633831_500000_CN_261185002_500000/RConn3 -- T_261185002__/LConn3 -- _CN_261185002_500000_CN_264410236_500000/RConn3 -- bus212/LConn1
  G_195105317_/RConn1 -- _CN_166633831_500000_CN_195105317_500000/RConn1
  G_195105317_/RConn2 -- _CN_166633831_500000_CN_195105317_500000/RConn2
  _CN_166633831_500000_CN_195105317_500000/RConn3 -- G_195105317_/RConn3 -- bus213/LConn1
  T_268532907__/RConn1 -- L_268532907/LConn1
  T_268532907__/RConn2 -- L_268532907/LConn2
  L_268532907/LConn3 -- T_268532907__/RConn3 -- bus214/LConn1
  T_268532908__/RConn1 -- L_268532908/LConn1
  T_268532908__/RConn2 -- L_268532908/LConn2
  L_268532908/LConn3 -- T_268532908__/RConn3 -- bus215/LConn1
  T_399277121__/RConn1 -- L_399277121/LConn1
  T_399277121__/RConn2 -- L_399277121/LConn2
  L_399277121/LConn3 -- T_399277121__/RConn3 -- bus216/LConn1
  T_261381125__/RConn1 -- L_261381125/LConn1
  T_261381125__/RConn2 -- L_261381125/LConn2
  L_261381125/LConn3 -- T_261381125__/RConn3 -- bus217/LConn1
  T_264719089__/RConn1 -- L_264719089/LConn1
  T_264719089__/RConn2 -- L_264719089/LConn2
  L_264719089/LConn3 -- T_264719089__/RConn3 -- bus218/LConn1
  T_264072199__/RConn1 -- L_264072199/LConn1
  T_264072199__/RConn2 -- L_264072199/LConn2
  L_264072199/LConn3 -- T_264072199__/RConn3 -- bus219/LConn1
  T_399057172__/RConn1 -- L_399057172/LConn1
  T_399057172__/RConn2 -- L_399057172/LConn2
  L_399057172/LConn3 -- T_399057172__/RConn3 -- bus220/LConn1
  T_186634762__/RConn1 -- L_186634762/LConn1
  T_186634762__/RConn2 -- L_186634762/LConn2
